simulink model "gm_MATE_HDLsolver_myFirstCircuit"  (R2024b)
settings: Solver=FixedStepDiscrete  StartTime=0.0  StopTime=0.05  FixedStep=6.02409638554217e-09  MaxStep=100e-6  RelTol=1e-4
PostLoadFcn:
  | Ts=1e-6; nb_sw=3; nb_lc=2;nb_r=1;nb_src=1; nb_out=3; rL=1.2;rC=100;L=1e-3; C=1e-5; LpejoSw=1e-6;h=Ts; MAX_INPUTS=16;
  | MAX_OUTPUTS=16;
  | MAX_SWITCHES=8;
  | MAX_INPUTS=16;
InitFcn:
  | Ts=1e-6; nb_sw=3; nb_lc=2;nb_r=1;nb_src=1; nb_out=3; rL=1.2;rC=100;L=1e-3; C=1e-5; LpejoSw=1e-6;h=Ts; MAX_INPUTS=16;
  | MAX_OUTPUTS=16;
  | MAX_SWITCHES=8;
  | MAX_INPUTS=16;
undefined symbols (not defined in the file or in its folder): MATE_SOC
libraries: fl_lib x31, nesl_utility x13, hdlmdlgenlib x10, simetranss x5, simulink x4, hdlsllib x3, ee_lib x2, eeGeneralControl x1
(part 2 of 8)

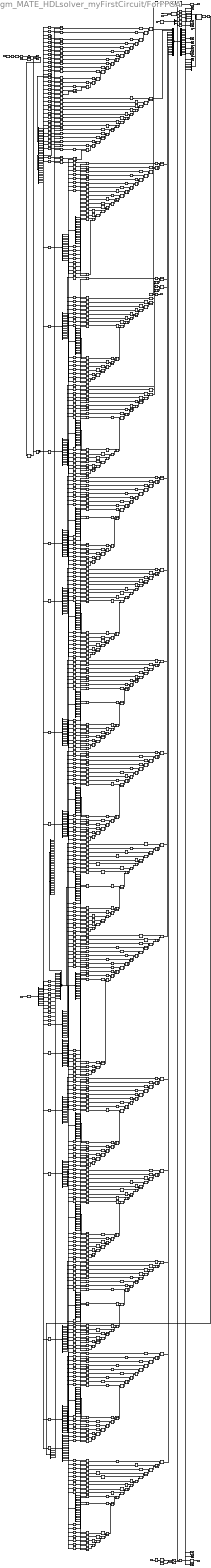
== system gm_MATE_HDLsolver_myFirstCircuit/ForFPGA ==
  note: Pejos
  mi : Inport  OutDataTypeStr=single  PortDimensions=1  SampleTime=1e-06
  PWMsteps : Inport  Port=2  OutDataTypeStr=uint16  PortDimensions=1  SampleTime=1e-06
  gate : Inport  Port=3  OutDataTypeStr=boolean  PortDimensions=[3]  SampleTime=1e-06
  minus_g : Inport  Port=4  OutDataTypeStr=single  PortDimensions=[5]  SampleTime=1e-06
  CrossIC : Inport  Port=5  OutDataTypeStr=boolean  PortDimensions=[5]  SampleTime=1e-06
  CrossICidx : Inport  Port=6  OutDataTypeStr=uint16  PortDimensions=[5]  SampleTime=1e-06
  D : Inport  Port=7  OutDataTypeStr=single  PortDimensions=1  SampleTime=1e-06
  Dcnt : Inport  Port=8  OutDataTypeStr=uint8  PortDimensions=1  SampleTime=1e-06
  in : Inport  Port=9  OutDataTypeStr=single  PortDimensions=[11]  SampleTime=1e-06
  out_start_range : Inport  Port=10  OutDataTypeStr=uint8  PortDimensions=1  SampleTime=1e-06
  Compare To Constant : Subsystem  mask(Compare To Constant){relop===, const=double(0), OutDataTypeStr=boolean, ZeroCross=on}
      mask prompts: relop "Simulink:masks:Operator_MP"; const "Simulink:masks:ConstantValue_MP"; OutDataTypeStr "Simulink:masks:OutputDataType_MP"; ZeroCross "Simulink:masks:EnableZerocrossingDetection_MP"
      mask help: Simulink:masks:CompareToConstant_MD
      mask init:
      | OutDataTypeStr = 'boolean';
      | ZeroCross = 'on';
      | blkName = 'MATE_HDLsolver_myFirstCircuit/ForFPGA/Compare\nTo Constant';
      | const = double(0);
      | const_str = '0';
      | const_val = double(0);
      | relop = '==';
      | setValue = 'boolean';
      | str = '== 0';
      mask TypeOptions relop: == | ~= | < | <= | >= | >
      mask TypeOptions OutDataTypeStr: Simulink:masks:uint8 | Simulink:masks:boolean
      mask Callback ZeroCross: sl('zeroCrossEnable', gcbh);
      mask Display: disp(str)
  Counter Free-Running : Subsystem  mask(Counter Free-Running){NumBits=double(4), tsamp=double(-1)}
      mask prompts: NumBits "Simulink:masks:NumberOfBits_MP"; tsamp "Simulink:masks:SampleTime_MP"
      mask help: Simulink:masks:CounterFreeRunning_MD
  Data Type Conversion1 : DataTypeConversion  OutDataTypeStr=boolean
  Data Type Conversion2 : DataTypeConversion  OutDataTypeStr=boolean
  Delay : RateTransition  InitialCondition=double(0)  OutPortSampleTimeOpt=Multiple of input port sample time  OutPortSampleTimeMultiple=166
  Delay_Switch : Switch  Criteria=u2 ~= 0  Threshold=double(0)  OutDataTypeStr=single  SampleTime=1e-06  SaturateOnIntegerOverflow=off  InputSameDT=off
  Delay_absorbed : Delay  DelayLength=0
  Demux_mux_1 : Mux  Inputs=5
  Dot Product : Subsystem
      mask Display: disp('NFP\nadd');
  Dot Product1 : Subsystem
      mask Display: disp('NFP\nadd');
  Dot Product10 : Subsystem
      mask Display: disp('NFP\nadd');
  Dot Product101 : Subsystem
      mask Display: disp('NFP\nadd');
  Dot Product1010 : Subsystem
      mask Display: disp('NFP\nadd');
  Dot Product1011 : Subsystem
      mask Display: disp('NFP\nadd');
  Dot Product1012 : Subsystem
      mask Display: disp('NFP\nadd');
  Dot Product1013 : Subsystem
      mask Display: disp('NFP\nadd');
  Dot Product1014 : Subsystem
      mask Display: disp('NFP\nadd');
  Dot Product1015 : Subsystem
      mask Display: disp('NFP\nadd');
  Dot Product102 : Subsystem
      mask Display: disp('NFP\nadd');
  Dot Product103 : Subsystem
      mask Display: disp('NFP\nadd');
  Dot Product104 : Subsystem
      mask Display: disp('NFP\nadd');
  Dot Product105 : Subsystem
      mask Display: disp('NFP\nadd');
  Dot Product106 : Subsystem
      mask Display: disp('NFP\nadd');
  Dot Product107 : Subsystem
      mask Display: disp('NFP\nadd');
  Dot Product108 : Subsystem
      mask Display: disp('NFP\nadd');
  Dot Product109 : Subsystem
      mask Display: disp('NFP\nadd');
  Dot Product11 : Subsystem
      mask Display: disp('NFP\nadd');
  Dot Product110 : Subsystem
      mask Display: disp('NFP\nadd');
  Dot Product111 : Subsystem
      mask Display: disp('NFP\nadd');
  Dot Product1110 : Subsystem
      mask Display: disp('NFP\nadd');
  Dot Product1111 : Subsystem
      mask Display: disp('NFP\nadd');
  Dot Product1112 : Subsystem
      mask Display: disp('NFP\nadd');
  Dot Product1113 : Subsystem
      mask Display: disp('NFP\nadd');
  Dot Product1114 : Subsystem
      mask Display: disp('NFP\nadd');
  Dot Product1115 : Subsystem
      mask Display: disp('NFP\nadd');
  Dot Product1116 : Subsystem
      mask Display: disp('NFP\nadd');
  Dot Product1117 : Subsystem
      mask Display: disp('NFP\nadd');
  Dot Product1118 : Subsystem
      mask Display: disp('NFP\nadd');
  Dot Product1119 : Subsystem
      mask Display: disp('NFP\nadd');
  Dot Product112 : Subsystem
      mask Display: disp('NFP\nadd');
  Dot Product1120 : Subsystem
      mask Display: disp('NFP\nadd');
  Dot Product1121 : Subsystem
      mask Display: disp('NFP\nadd');
  Dot Product1122 : Subsystem
      mask Display: disp('NFP\nadd');
  Dot Product1123 : Subsystem
      mask Display: disp('NFP\nadd');
  Dot Product1124 : Subsystem
      mask Display: disp('NFP\nadd');
  Dot Product113 : Subsystem
      mask Display: disp('NFP\nadd');
  Dot Product114 : Subsystem
      mask Display: disp('NFP\nadd');
  Dot Product115 : Subsystem
      mask Display: disp('NFP\nadd');
  Dot Product116 : Subsystem
      mask Display: disp('NFP\nadd');
  Dot Product117 : Subsystem
      mask Display: disp('NFP\nadd');
  Dot Product118 : Subsystem
      mask Display: disp('NFP\nadd');
  Dot Product119 : Subsystem
      mask Display: disp('NFP\nadd');
  Dot Product12 : Subsystem
      mask Display: disp('NFP\nadd');
  Dot Product121 : Subsystem
      mask Display: disp('NFP\nadd');
  Dot Product1210 : Subsystem
      mask Display: disp('NFP\nadd');
  Dot Product1211 : Subsystem
      mask Display: disp('NFP\nadd');
  Dot Product1212 : Subsystem
      mask Display: disp('NFP\nadd');
  Dot Product1213 : Subsystem
      mask Display: disp('NFP\nadd');
  Dot Product1214 : Subsystem
      mask Display: disp('NFP\nadd');
  Dot Product1215 : Subsystem
      mask Display: disp('NFP\nadd');
  Dot Product122 : Subsystem
      mask Display: disp('NFP\nadd');
  Dot Product123 : Subsystem
      mask Display: disp('NFP\nadd');
  Dot Product124 : Subsystem
      mask Display: disp('NFP\nadd');
  Dot Product125 : Subsystem
      mask Display: disp('NFP\nadd');
  Dot Product126 : Subsystem
      mask Display: disp('NFP\nadd');
  Dot Product127 : Subsystem
      mask Display: disp('NFP\nadd');
  Dot Product128 : Subsystem
      mask Display: disp('NFP\nadd');
  Dot Product129 : Subsystem
      mask Display: disp('NFP\nadd');
  Dot Product13 : Subsystem
      mask Display: disp('NFP\nadd');
  Dot Product131 : Subsystem
      mask Display: disp('NFP\nadd');
  Dot Product1310 : Subsystem
      mask Display: disp('NFP\nadd');
  Dot Product1311 : Subsystem
      mask Display: disp('NFP\nadd');
  Dot Product1312 : Subsystem
      mask Display: disp('NFP\nadd');
  Dot Product1313 : Subsystem
      mask Display: disp('NFP\nadd');
  Dot Product1314 : Subsystem
      mask Display: disp('NFP\nadd');
  Dot Product1315 : Subsystem
      mask Display: disp('NFP\nadd');
  Dot Product132 : Subsystem
      mask Display: disp('NFP\nadd');
  Dot Product133 : Subsystem
      mask Display: disp('NFP\nadd');
  Dot Product134 : Subsystem
      mask Display: disp('NFP\nadd');
  Dot Product135 : Subsystem
      mask Display: disp('NFP\nadd');
  Dot Product136 : Subsystem
      mask Display: disp('NFP\nadd');
  Dot Product137 : Subsystem
      mask Display: disp('NFP\nadd');
  Dot Product138 : Subsystem
      mask Display: disp('NFP\nadd');
  Dot Product139 : Subsystem
      mask Display: disp('NFP\nadd');
  Dot Product14 : Subsystem
      mask Display: disp('NFP\nadd');
  Dot Product141 : Subsystem
      mask Display: disp('NFP\nadd');
  Dot Product1410 : Subsystem
      mask Display: disp('NFP\nadd');
  Dot Product1411 : Subsystem
      mask Display: disp('NFP\nadd');
  Dot Product1412 : Subsystem
      mask Display: disp('NFP\nadd');
  Dot Product1413 : Subsystem
      mask Display: disp('NFP\nadd');
  Dot Product1414 : Subsystem
      mask Display: disp('NFP\nadd');
  Dot Product1415 : Subsystem
      mask Display: disp('NFP\nadd');
  Dot Product142 : Subsystem
      mask Display: disp('NFP\nadd');
  Dot Product143 : Subsystem
      mask Display: disp('NFP\nadd');
  Dot Product144 : Subsystem
      mask Display: disp('NFP\nadd');
  Dot Product145 : Subsystem
      mask Display: disp('NFP\nadd');
  Dot Product146 : Subsystem
      mask Display: disp('NFP\nadd');
  Dot Product147 : Subsystem
      mask Display: disp('NFP\nadd');
  Dot Product148 : Subsystem
      mask Display: disp('NFP\nadd');
  Dot Product149 : Subsystem
      mask Display: disp('NFP\nadd');
  Dot Product15 : Subsystem
      mask Display: disp('NFP\nadd');
  Dot Product151 : Subsystem
      mask Display: disp('NFP\nadd');
  Dot Product1510 : Subsystem
      mask Display: disp('NFP\nadd');
  Dot Product1511 : Subsystem
      mask Display: disp('NFP\nadd');
  Dot Product1512 : Subsystem
      mask Display: disp('NFP\nadd');
  Dot Product1513 : Subsystem
      mask Display: disp('NFP\nadd');
  Dot Product1514 : Subsystem
      mask Display: disp('NFP\nadd');
  Dot Product1515 : Subsystem
      mask Display: disp('NFP\nadd');
  Dot Product152 : Subsystem
      mask Display: disp('NFP\nadd');
  Dot Product153 : Subsystem
      mask Display: disp('NFP\nadd');
  Dot Product154 : Subsystem
      mask Display: disp('NFP\nadd');
  Dot Product155 : Subsystem
      mask Display: disp('NFP\nadd');
  Dot Product156 : Subsystem
      mask Display: disp('NFP\nadd');
  Dot Product157 : Subsystem
      mask Display: disp('NFP\nadd');
  Dot Product158 : Subsystem
      mask Display: disp('NFP\nadd');
  Dot Product159 : Subsystem
      mask Display: disp('NFP\nadd');
  Dot Product16 : Subsystem
      mask Display: disp('NFP\nadd');
  Dot Product17 : Subsystem
      mask Display: disp('NFP\nadd');
  Dot Product18 : Subsystem
      mask Display: disp('NFP\nadd');
  Dot Product19 : Subsystem
      mask Display: disp('NFP\nadd');
  Dot Product2 : Subsystem
      mask Display: disp('NFP\nadd');
  Dot Product21 : Subsystem
      mask Display: disp('NFP\nadd');
  Dot Product210 : Subsystem
      mask Display: disp('NFP\nadd');
  Dot Product211 : Subsystem
      mask Display: disp('NFP\nadd');
  Dot Product212 : Subsystem
      mask Display: disp('NFP\nadd');
  Dot Product213 : Subsystem
      mask Display: disp('NFP\nadd');
  Dot Product214 : Subsystem
      mask Display: disp('NFP\nadd');
  Dot Product215 : Subsystem
      mask Display: disp('NFP\nadd');
  Dot Product22 : Subsystem
      mask Display: disp('NFP\nadd');
  Dot Product23 : Subsystem
      mask Display: disp('NFP\nadd');
  Dot Product24 : Subsystem
      mask Display: disp('NFP\nadd');
  Dot Product25 : Subsystem
      mask Display: disp('NFP\nadd');
  Dot Product26 : Subsystem
      mask Display: disp('NFP\nadd');
  Dot Product27 : Subsystem
      mask Display: disp('NFP\nadd');
  Dot Product28 : Subsystem
      mask Display: disp('NFP\nadd');
  Dot Product29 : Subsystem
      mask Display: disp('NFP\nadd');
  Dot Product3 : Subsystem
      mask Display: disp('NFP\nadd');
  Dot Product31 : Subsystem
      mask Display: disp('NFP\nadd');
  Dot Product310 : Subsystem
      mask Display: disp('NFP\nadd');
  Dot Product311 : Subsystem
      mask Display: disp('NFP\nadd');
  Dot Product312 : Subsystem
      mask Display: disp('NFP\nadd');
  Dot Product313 : Subsystem
      mask Display: disp('NFP\nadd');
  Dot Product314 : Subsystem
      mask Display: disp('NFP\nadd');
  Dot Product315 : Subsystem
      mask Display: disp('NFP\nadd');
  Dot Product32 : Subsystem
      mask Display: disp('NFP\nadd');
  Dot Product33 : Subsystem
      mask Display: disp('NFP\nadd');
  Dot Product34 : Subsystem
      mask Display: disp('NFP\nadd');
  Dot Product35 : Subsystem
      mask Display: disp('NFP\nadd');
  Dot Product36 : Subsystem
      mask Display: disp('NFP\nadd');
  Dot Product37 : Subsystem
      mask Display: disp('NFP\nadd');
  Dot Product38 : Subsystem
      mask Display: disp('NFP\nadd');
  Dot Product39 : Subsystem
      mask Display: disp('NFP\nadd');
  Dot Product4 : Subsystem
      mask Display: disp('NFP\nadd');
  Dot Product41 : Subsystem
      mask Display: disp('NFP\nadd');
  Dot Product410 : Subsystem
      mask Display: disp('NFP\nadd');
  Dot Product411 : Subsystem
      mask Display: disp('NFP\nadd');
  Dot Product412 : Subsystem
      mask Display: disp('NFP\nadd');
  Dot Product413 : Subsystem
      mask Display: disp('NFP\nadd');
  Dot Product414 : Subsystem
      mask Display: disp('NFP\nadd');
  Dot Product415 : Subsystem
      mask Display: disp('NFP\nadd');
  Dot Product42 : Subsystem
      mask Display: disp('NFP\nadd');
  Dot Product43 : Subsystem
      mask Display: disp('NFP\nadd');
  Dot Product44 : Subsystem
      mask Display: disp('NFP\nadd');
  Dot Product45 : Subsystem
      mask Display: disp('NFP\nadd');
  Dot Product46 : Subsystem
      mask Display: disp('NFP\nadd');
  Dot Product47 : Subsystem
      mask Display: disp('NFP\nadd');
  Dot Product48 : Subsystem
      mask Display: disp('NFP\nadd');
  Dot Product49 : Subsystem
      mask Display: disp('NFP\nadd');
  Dot Product5 : Subsystem
      mask Display: disp('NFP\nadd');
  Dot Product51 : Subsystem
      mask Display: disp('NFP\nadd');
  Dot Product510 : Subsystem
      mask Display: disp('NFP\nadd');
  Dot Product511 : Subsystem
      mask Display: disp('NFP\nadd');
  Dot Product512 : Subsystem
      mask Display: disp('NFP\nadd');
  Dot Product513 : Subsystem
      mask Display: disp('NFP\nadd');
  Dot Product514 : Subsystem
      mask Display: disp('NFP\nadd');
  Dot Product515 : Subsystem
      mask Display: disp('NFP\nadd');
  Dot Product52 : Subsystem
      mask Display: disp('NFP\nadd');
  Dot Product53 : Subsystem
      mask Display: disp('NFP\nadd');
  Dot Product54 : Subsystem
      mask Display: disp('NFP\nadd');
  Dot Product55 : Subsystem
      mask Display: disp('NFP\nadd');
  Dot Product56 : Subsystem
      mask Display: disp('NFP\nadd');
  Dot Product57 : Subsystem
      mask Display: disp('NFP\nadd');
  Dot Product58 : Subsystem
      mask Display: disp('NFP\nadd');
  Dot Product59 : Subsystem
      mask Display: disp('NFP\nadd');
  Dot Product6 : Subsystem
      mask Display: disp('NFP\nadd');
  Dot Product61 : Subsystem
      mask Display: disp('NFP\nadd');
  Dot Product610 : Subsystem
      mask Display: disp('NFP\nadd');
  Dot Product611 : Subsystem
      mask Display: disp('NFP\nadd');
  Dot Product612 : Subsystem
      mask Display: disp('NFP\nadd');
  Dot Product613 : Subsystem
      mask Display: disp('NFP\nadd');
  Dot Product614 : Subsystem
      mask Display: disp('NFP\nadd');
  Dot Product615 : Subsystem
      mask Display: disp('NFP\nadd');
  Dot Product62 : Subsystem
      mask Display: disp('NFP\nadd');
  Dot Product63 : Subsystem
      mask Display: disp('NFP\nadd');
  Dot Product64 : Subsystem
      mask Display: disp('NFP\nadd');
  Dot Product65 : Subsystem
      mask Display: disp('NFP\nadd');
  Dot Product66 : Subsystem
      mask Display: disp('NFP\nadd');
  Dot Product67 : Subsystem
      mask Display: disp('NFP\nadd');
  Dot Product68 : Subsystem
      mask Display: disp('NFP\nadd');
  Dot Product69 : Subsystem
      mask Display: disp('NFP\nadd');
  Dot Product7 : Subsystem
      mask Display: disp('NFP\nadd');
  Dot Product71 : Subsystem
      mask Display: disp('NFP\nadd');
  Dot Product710 : Subsystem
      mask Display: disp('NFP\nadd');
  Dot Product711 : Subsystem
      mask Display: disp('NFP\nadd');
  Dot Product712 : Subsystem
      mask Display: disp('NFP\nadd');
  Dot Product713 : Subsystem
      mask Display: disp('NFP\nadd');
  Dot Product714 : Subsystem
      mask Display: disp('NFP\nadd');
  Dot Product715 : Subsystem
      mask Display: disp('NFP\nadd');
  Dot Product72 : Subsystem
      mask Display: disp('NFP\nadd');
  Dot Product73 : Subsystem
      mask Display: disp('NFP\nadd');
  Dot Product74 : Subsystem
      mask Display: disp('NFP\nadd');
  Dot Product75 : Subsystem
      mask Display: disp('NFP\nadd');
  Dot Product76 : Subsystem
      mask Display: disp('NFP\nadd');
  Dot Product77 : Subsystem
      mask Display: disp('NFP\nadd');
  Dot Product78 : Subsystem
      mask Display: disp('NFP\nadd');
  Dot Product79 : Subsystem
      mask Display: disp('NFP\nadd');
  Dot Product8 : Subsystem
      mask Display: disp('NFP\nadd');
  Dot Product81 : Subsystem
      mask Display: disp('NFP\nadd');
  Dot Product810 : Subsystem
      mask Display: disp('NFP\nadd');
  Dot Product811 : Subsystem
      mask Display: disp('NFP\nadd');
  Dot Product812 : Subsystem
      mask Display: disp('NFP\nadd');
  Dot Product813 : Subsystem
      mask Display: disp('NFP\nadd');
  Dot Product814 : Subsystem
      mask Display: disp('NFP\nadd');
  Dot Product815 : Subsystem
      mask Display: disp('NFP\nadd');
  Dot Product82 : Subsystem
      mask Display: disp('NFP\nadd');
  Dot Product83 : Subsystem
      mask Display: disp('NFP\nadd');
  Dot Product84 : Subsystem
      mask Display: disp('NFP\nadd');
  Dot Product85 : Subsystem
      mask Display: disp('NFP\nadd');
  Dot Product86 : Subsystem
      mask Display: disp('NFP\nadd');
  Dot Product87 : Subsystem
      mask Display: disp('NFP\nadd');
  Dot Product88 : Subsystem
      mask Display: disp('NFP\nadd');
  Dot Product89 : Subsystem
      mask Display: disp('NFP\nadd');
  Dot Product9 : Subsystem
      mask Display: disp('NFP\nadd');
  Dot Product91 : Subsystem
      mask Display: disp('NFP\nadd');
  Dot Product910 : Subsystem
      mask Display: disp('NFP\nadd');
  Dot Product911 : Subsystem
      mask Display: disp('NFP\nadd');
  Dot Product912 : Subsystem
      mask Display: disp('NFP\nadd');
  Dot Product913 : Subsystem
      mask Display: disp('NFP\nadd');
  Dot Product914 : Subsystem
      mask Display: disp('NFP\nadd');
  Dot Product915 : Subsystem
      mask Display: disp('NFP\nadd');
  Dot Product92 : Subsystem
      mask Display: disp('NFP\nadd');
  Dot Product93 : Subsystem
      mask Display: disp('NFP\nadd');
  Dot Product94 : Subsystem
      mask Display: disp('NFP\nadd');
  Dot Product95 : Subsystem
      mask Display: disp('NFP\nadd');
  Dot Product96 : Subsystem
      mask Display: disp('NFP\nadd');
  Dot Product97 : Subsystem
      mask Display: disp('NFP\nadd');
  Dot Product98 : Subsystem
      mask Display: disp('NFP\nadd');
  Dot Product99 : Subsystem
      mask Display: disp('NFP\nadd');
  From : hdlmdlgenlib/Buffer
  Goto : hdlmdlgenlib/Buffer
  Index Vector : MultiPortSwitch  DataPortOrder=Zero-based contiguous  Inputs=1  DiagnosticForDefault=None  zeroidx=on  OutDataTypeStr=single  SampleTime=6.02409638554217e-09  SaturateOnIntegerOverflow=off  InputSameDT=off
  Index Vector_dtc_comp : DataTypeConversion  OutDataTypeStr=fixdt(0, 4, 0)  SampleTime=6.02409638554217e-09  SaturateOnIntegerOverflow=off
  LC vectorized : Subsystem
  Mux4_out1_10_term10 : Terminator
  Mux4_out1_11_term11 : Terminator
  Mux4_out1_12_term12 : Terminator
  Mux4_out1_13_term13 : Terminator
  Mux4_out1_14_term14 : Terminator
  Mux4_out1_15_term15 : Terminator
  Mux4_out1_5_term5 : Terminator
  Mux4_out1_6_term6 : Terminator
  Mux4_out1_7_term7 : Terminator
  Mux4_out1_8_term8 : Terminator
  Mux4_out1_9_term9 : Terminator
  PWM Generator : Subsystem
  Selector : Selector  InputPortWidth=256  IndexOptions=Index vector (dialog)  Indices=double([1 2 3 4 5 6 7 8 9 10 11 12 13 14 15 16])  OutputSizes=double(1)
  Selector1 : Selector  InputPortWidth=256  IndexOptions=Index vector (dialog)  Indices=double([17 18 19 20 21 22 23 24 25 26 27 28 29 30 31 32])  OutputSizes=double(1)
  Selector10 : Selector  InputPortWidth=256  IndexOptions=Index vector (dialog)  Indices=double([161 162 163 164 165 166 167 168 169 170 171 172 173 174 175 176])  OutputSizes=double(1)
  Selector11 : Selector  InputPortWidth=256  IndexOptions=Index vector (dialog)  Indices=double([177 178 179 180 181 182 183 184 185 186 187 188 189 190 191 192])  OutputSizes=double(1)
  Selector12 : Selector  InputPortWidth=256  IndexOptions=Index vector (dialog)  Indices=double([193 194 195 196 197 198 199 200 201 202 203 204 205 206 207 208])  OutputSizes=double(1)
  Selector13 : Selector  InputPortWidth=256  IndexOptions=Index vector (dialog)  Indices=double([209 210 211 212 213 214 215 216 217 218 219 220 221 222 223 224])  OutputSizes=double(1)
  Selector14 : Selector  InputPortWidth=256  IndexOptions=Index vector (dialog)  Indices=double([225 226 227 228 229 230 231 232 233 234 235 236 237 238 239 240])  OutputSizes=double(1)
  Selector15 : Selector  InputPortWidth=256  IndexOptions=Index vector (dialog)  Indices=double([241 242 243 244 245 246 247 248 249 250 251 252 253 254 255 256])  OutputSizes=double(1)
  Selector16 : Selector  InputPortWidth=16  IndexOptions=Starting index (port)  Indices=double([1 2 3 4 5 6 7 8 9 10 11 12 13 14 15 16])  OutputSizes=double(8)
  Selector2 : Selector  InputPortWidth=256  IndexOptions=Index vector (dialog)  Indices=double([33 34 35 36 37 38 39 40 41 42 43 44 45 46 47 48])  OutputSizes=double(1)
  Selector3 : Selector  InputPortWidth=256  IndexOptions=Index vector (dialog)  Indices=double([49 50 51 52 53 54 55 56 57 58 59 60 61 62 63 64])  OutputSizes=double(1)
  Selector4 : Selector  InputPortWidth=256  IndexOptions=Index vector (dialog)  Indices=double([65 66 67 68 69 70 71 72 73 74 75 76 77 78 79 80])  OutputSizes=double(1)
  Selector5 : Selector  InputPortWidth=256  IndexOptions=Index vector (dialog)  Indices=double([81 82 83 84 85 86 87 88 89 90 91 92 93 94 95 96])  OutputSizes=double(1)
  Selector6 : Selector  InputPortWidth=256  IndexOptions=Index vector (dialog)  Indices=double([97 98 99 100 101 102 103 104 105 106 107 108 109 110 111 112])  OutputSizes=double(1)
  Selector7 : Selector  InputPortWidth=256  IndexOptions=Index vector (dialog)  Indices=double([113 114 115 116 117 118 119 120 121 122 123 124 125 126 127 128])  OutputSizes=double(1)
  Selector8 : Selector  InputPortWidth=256  IndexOptions=Index vector (dialog)  Indices=double([129 130 131 132 133 134 135 136 137 138 139 140 141 142 143 144])  OutputSizes=double(1)
  Selector9 : Selector  InputPortWidth=256  IndexOptions=Index vector (dialog)  Indices=double([145 146 147 148 149 150 151 152 153 154 155 156 157 158 159 160])  OutputSizes=double(1)
  Tapped Delay : simulink/Discrete/Tapped Delay  vinit=0  samptime=-1  NumDelays=double(255)  DelayOrder=Oldest  includeCurrent=on
  Unit Delay Enabled Synchronous22_lowered : Delay  DelayLength=double(1)  InitialCondition=0  SampleTime=1e-06
  crp_out_delay : Delay  DelayLength=double(1)  InitialCondition=0  SampleTime=6.02409638554217e-09
  delayMatch{,1..29,33,44..59,63,74..89,93,104..119,123,134..149,153,164..179,183,194..209,213,224..239,243,254..269,273,284..299,303,314..329,333,344..359,363,374..389,393,404..419,423,434..449,453,464..479,483} (286 alike) : Delay  DelayLength=double(24)  InitialCondition=0  SampleTime=6.02409638554217e-09
  delayMatch{40,70,100,130,160,190,220,250,280,310,340,370,400,430,460,490} (16 alike) : Delay  DelayLength=double(66)  InitialCondition=0  SampleTime=6.02409638554217e-09
  delayMatch{41,71,101,131,161,191,221,251,281,311,341,371,401,431,461,491} (16 alike) : Delay  DelayLength=double(72)  InitialCondition=0  SampleTime=6.02409638554217e-09
  delayMatch{42,72,102,132,162,192,222,252,282,312,342,372,402,432,462,492} (16 alike) : Delay  DelayLength=double(78)  InitialCondition=0  SampleTime=6.02409638554217e-09
  delayMatch{43,73,103,133,163,193,223,253,283,313,343,373,403,433,463,493} (16 alike) : Delay  DelayLength=double(84)  InitialCondition=0  SampleTime=6.02409638554217e-09
  delayMatch{30,60,90,120,150,180,210,240,270,300,330,360,390,420,450,480} (16 alike) : Delay  DelayLength=double(6)  InitialCondition=0  SampleTime=6.02409638554217e-09
  delayMatch{31,61,91,121,151,181,211,241,271,301,331,361,391,421,451,481} (16 alike) : Delay  DelayLength=double(12)  InitialCondition=0  SampleTime=6.02409638554217e-09
  delayMatch{32,62,92,122,152,182,212,242,272,302,332,362,392,422,452,482} (16 alike) : Delay  DelayLength=double(18)  InitialCondition=0  SampleTime=6.02409638554217e-09
  delayMatch{34,64,94,124,154,184,214,244,274,304,334,364,394,424,454,484} (16 alike) : Delay  DelayLength=double(30)  InitialCondition=0  SampleTime=6.02409638554217e-09
  delayMatch{35,65,95,125,155,185,215,245,275,305,335,365,395,425,455,485} (16 alike) : Delay  DelayLength=double(36)  InitialCondition=0  SampleTime=6.02409638554217e-09
  delayMatch{36,66,96,126,156,186,216,246,276,306,336,366,396,426,456,486} (16 alike) : Delay  DelayLength=double(42)  InitialCondition=0  SampleTime=6.02409638554217e-09
  delayMatch{37,67,97,127,157,187,217,247,277,307,337,367,397,427,457,487} (16 alike) : Delay  DelayLength=double(48)  InitialCondition=0  SampleTime=6.02409638554217e-09
  delayMatch{38,68,98,128,158,188,218,248,278,308,338,368,398,428,458,488} (16 alike) : Delay  DelayLength=double(54)  InitialCondition=0  SampleTime=6.02409638554217e-09
  delayMatch{39,69,99,129,159,189,219,249,279,309,339,369,399,429,459,489} (16 alike) : Delay  DelayLength=double(60)  InitialCondition=0  SampleTime=6.02409638554217e-09
  delayMatch494 : Delay  DelayLength=double(1)  InitialCondition=0  SampleTime=6.02409638554217e-09
  delayMatch495 : Delay  DelayLength=double(1)  InitialCondition=0  SampleTime=6.02409638554217e-09
  delayMatch496 : Delay  DelayLength=double(1)  InitialCondition=0  SampleTime=1e-06
  in0_repeat : RateTransition  Integrity=off  Deterministic=off  OutPortSampleTimeOpt=Multiple of input port sample time  OutPortSampleTimeMultiple=1/166
  in1_repeat : RateTransition  Integrity=off  Deterministic=off  OutPortSampleTimeOpt=Multiple of input port sample time  OutPortSampleTimeMultiple=1/166
  in2_repeat : RateTransition  Integrity=off  Deterministic=off  OutPortSampleTimeOpt=Multiple of input port sample time  OutPortSampleTimeMultiple=1/166
  in3_repeat : RateTransition  Integrity=off  Deterministic=off  OutPortSampleTimeOpt=Multiple of input port sample time  OutPortSampleTimeMultiple=1/166
  in3_repeat1 : RateTransition  Integrity=off  Deterministic=off  OutPortSampleTimeOpt=Multiple of input port sample time  OutPortSampleTimeMultiple=1/166
  in4_repeat : RateTransition  Integrity=off  Deterministic=off  OutPortSampleTimeOpt=Multiple of input port sample time  OutPortSampleTimeMultiple=1/166
  mul_Dot Product10_dotp_0 : Subsystem
      mask Display: disp('NFP\nmul');
  mul_Dot Product10_dotp_1 : Subsystem
      mask Display: disp('NFP\nmul');
  mul_Dot Product10_dotp_10 : Subsystem
      mask Display: disp('NFP\nmul');
  mul_Dot Product10_dotp_11 : Subsystem
      mask Display: disp('NFP\nmul');
  mul_Dot Product10_dotp_12 : Subsystem
      mask Display: disp('NFP\nmul');
  mul_Dot Product10_dotp_13 : Subsystem
      mask Display: disp('NFP\nmul');
  mul_Dot Product10_dotp_14 : Subsystem
      mask Display: disp('NFP\nmul');
  mul_Dot Product10_dotp_15 : Subsystem
      mask Display: disp('NFP\nmul');
  mul_Dot Product10_dotp_2 : Subsystem
      mask Display: disp('NFP\nmul');
  mul_Dot Product10_dotp_3 : Subsystem
      mask Display: disp('NFP\nmul');
  mul_Dot Product10_dotp_4 : Subsystem
      mask Display: disp('NFP\nmul');
  mul_Dot Product10_dotp_5 : Subsystem
      mask Display: disp('NFP\nmul');
  mul_Dot Product10_dotp_6 : Subsystem
      mask Display: disp('NFP\nmul');
  mul_Dot Product10_dotp_7 : Subsystem
      mask Display: disp('NFP\nmul');
  mul_Dot Product10_dotp_8 : Subsystem
      mask Display: disp('NFP\nmul');
  mul_Dot Product10_dotp_9 : Subsystem
      mask Display: disp('NFP\nmul');
  mul_Dot Product11_dotp_0 : Subsystem
      mask Display: disp('NFP\nmul');
  mul_Dot Product11_dotp_1 : Subsystem
      mask Display: disp('NFP\nmul');
  mul_Dot Product11_dotp_10 : Subsystem
      mask Display: disp('NFP\nmul');
  mul_Dot Product11_dotp_11 : Subsystem
      mask Display: disp('NFP\nmul');
  mul_Dot Product11_dotp_12 : Subsystem
      mask Display: disp('NFP\nmul');
  mul_Dot Product11_dotp_13 : Subsystem
      mask Display: disp('NFP\nmul');
  mul_Dot Product11_dotp_14 : Subsystem
      mask Display: disp('NFP\nmul');
  mul_Dot Product11_dotp_15 : Subsystem
      mask Display: disp('NFP\nmul');
  mul_Dot Product11_dotp_2 : Subsystem
      mask Display: disp('NFP\nmul');
  mul_Dot Product11_dotp_3 : Subsystem
      mask Display: disp('NFP\nmul');
  mul_Dot Product11_dotp_4 : Subsystem
      mask Display: disp('NFP\nmul');
  mul_Dot Product11_dotp_5 : Subsystem
      mask Display: disp('NFP\nmul');
  mul_Dot Product11_dotp_6 : Subsystem
      mask Display: disp('NFP\nmul');
  mul_Dot Product11_dotp_7 : Subsystem
      mask Display: disp('NFP\nmul');
  mul_Dot Product11_dotp_8 : Subsystem
      mask Display: disp('NFP\nmul');
  mul_Dot Product11_dotp_9 : Subsystem
      mask Display: disp('NFP\nmul');
  mul_Dot Product12_dotp_0 : Subsystem
      mask Display: disp('NFP\nmul');
  mul_Dot Product12_dotp_1 : Subsystem
      mask Display: disp('NFP\nmul');
  mul_Dot Product12_dotp_10 : Subsystem
      mask Display: disp('NFP\nmul');
  mul_Dot Product12_dotp_11 : Subsystem
      mask Display: disp('NFP\nmul');
  mul_Dot Product12_dotp_12 : Subsystem
      mask Display: disp('NFP\nmul');
  mul_Dot Product12_dotp_13 : Subsystem
      mask Display: disp('NFP\nmul');
  mul_Dot Product12_dotp_14 : Subsystem
      mask Display: disp('NFP\nmul');
  mul_Dot Product12_dotp_15 : Subsystem
      mask Display: disp('NFP\nmul');
  mul_Dot Product12_dotp_2 : Subsystem
      mask Display: disp('NFP\nmul');
  mul_Dot Product12_dotp_3 : Subsystem
      mask Display: disp('NFP\nmul');
  mul_Dot Product12_dotp_4 : Subsystem
      mask Display: disp('NFP\nmul');
  mul_Dot Product12_dotp_5 : Subsystem
      mask Display: disp('NFP\nmul');
  mul_Dot Product12_dotp_6 : Subsystem
      mask Display: disp('NFP\nmul');
  mul_Dot Product12_dotp_7 : Subsystem
      mask Display: disp('NFP\nmul');
  mul_Dot Product12_dotp_8 : Subsystem
      mask Display: disp('NFP\nmul');
  mul_Dot Product12_dotp_9 : Subsystem
      mask Display: disp('NFP\nmul');
  mul_Dot Product13_dotp_0 : Subsystem
      mask Display: disp('NFP\nmul');
  mul_Dot Product13_dotp_1 : Subsystem
      mask Display: disp('NFP\nmul');
  mul_Dot Product13_dotp_10 : Subsystem
      mask Display: disp('NFP\nmul');
  mul_Dot Product13_dotp_11 : Subsystem
      mask Display: disp('NFP\nmul');
  mul_Dot Product13_dotp_12 : Subsystem
      mask Display: disp('NFP\nmul');
  mul_Dot Product13_dotp_13 : Subsystem
      mask Display: disp('NFP\nmul');
  mul_Dot Product13_dotp_14 : Subsystem
      mask Display: disp('NFP\nmul');
  mul_Dot Product13_dotp_15 : Subsystem
      mask Display: disp('NFP\nmul');
  mul_Dot Product13_dotp_2 : Subsystem
      mask Display: disp('NFP\nmul');
  mul_Dot Product13_dotp_3 : Subsystem
      mask Display: disp('NFP\nmul');
  mul_Dot Product13_dotp_4 : Subsystem
      mask Display: disp('NFP\nmul');
  mul_Dot Product13_dotp_5 : Subsystem
      mask Display: disp('NFP\nmul');
  mul_Dot Product13_dotp_6 : Subsystem
      mask Display: disp('NFP\nmul');
  mul_Dot Product13_dotp_7 : Subsystem
      mask Display: disp('NFP\nmul');
  mul_Dot Product13_dotp_8 : Subsystem
      mask Display: disp('NFP\nmul');
  mul_Dot Product13_dotp_9 : Subsystem
      mask Display: disp('NFP\nmul');
  mul_Dot Product14_dotp_0 : Subsystem
      mask Display: disp('NFP\nmul');
  mul_Dot Product14_dotp_1 : Subsystem
      mask Display: disp('NFP\nmul');
  mul_Dot Product14_dotp_10 : Subsystem
      mask Display: disp('NFP\nmul');
  mul_Dot Product14_dotp_11 : Subsystem
      mask Display: disp('NFP\nmul');
  mul_Dot Product14_dotp_12 : Subsystem
      mask Display: disp('NFP\nmul');
  mul_Dot Product14_dotp_13 : Subsystem
      mask Display: disp('NFP\nmul');
  mul_Dot Product14_dotp_14 : Subsystem
      mask Display: disp('NFP\nmul');
  mul_Dot Product14_dotp_15 : Subsystem
      mask Display: disp('NFP\nmul');
  mul_Dot Product14_dotp_2 : Subsystem
      mask Display: disp('NFP\nmul');
  mul_Dot Product14_dotp_3 : Subsystem
      mask Display: disp('NFP\nmul');
  mul_Dot Product14_dotp_4 : Subsystem
      mask Display: disp('NFP\nmul');
  mul_Dot Product14_dotp_5 : Subsystem
      mask Display: disp('NFP\nmul');
  mul_Dot Product14_dotp_6 : Subsystem
      mask Display: disp('NFP\nmul');
  mul_Dot Product14_dotp_7 : Subsystem
      mask Display: disp('NFP\nmul');
  mul_Dot Product14_dotp_8 : Subsystem
      mask Display: disp('NFP\nmul');
  mul_Dot Product14_dotp_9 : Subsystem
      mask Display: disp('NFP\nmul');
  mul_Dot Product15_dotp_0 : Subsystem
      mask Display: disp('NFP\nmul');
  mul_Dot Product15_dotp_1 : Subsystem
      mask Display: disp('NFP\nmul');
  mul_Dot Product15_dotp_10 : Subsystem
      mask Display: disp('NFP\nmul');
  mul_Dot Product15_dotp_11 : Subsystem
      mask Display: disp('NFP\nmul');
  mul_Dot Product15_dotp_12 : Subsystem
      mask Display: disp('NFP\nmul');
  mul_Dot Product15_dotp_13 : Subsystem
      mask Display: disp('NFP\nmul');
  mul_Dot Product15_dotp_14 : Subsystem
      mask Display: disp('NFP\nmul');
  mul_Dot Product15_dotp_15 : Subsystem
      mask Display: disp('NFP\nmul');
  mul_Dot Product15_dotp_2 : Subsystem
      mask Display: disp('NFP\nmul');
  mul_Dot Product15_dotp_3 : Subsystem
      mask Display: disp('NFP\nmul');
  mul_Dot Product15_dotp_4 : Subsystem
      mask Display: disp('NFP\nmul');
  mul_Dot Product15_dotp_5 : Subsystem
      mask Display: disp('NFP\nmul');
  mul_Dot Product15_dotp_6 : Subsystem
      mask Display: disp('NFP\nmul');
  mul_Dot Product15_dotp_7 : Subsystem
      mask Display: disp('NFP\nmul');
  mul_Dot Product15_dotp_8 : Subsystem
      mask Display: disp('NFP\nmul');
  mul_Dot Product15_dotp_9 : Subsystem
      mask Display: disp('NFP\nmul');
  mul_Dot Product1_dotp_0 : Subsystem
      mask Display: disp('NFP\nmul');
  mul_Dot Product1_dotp_1 : Subsystem
      mask Display: disp('NFP\nmul');
  mul_Dot Product1_dotp_10 : Subsystem
      mask Display: disp('NFP\nmul');
  mul_Dot Product1_dotp_11 : Subsystem
      mask Display: disp('NFP\nmul');
  mul_Dot Product1_dotp_12 : Subsystem
      mask Display: disp('NFP\nmul');
  mul_Dot Product1_dotp_13 : Subsystem
      mask Display: disp('NFP\nmul');
  mul_Dot Product1_dotp_14 : Subsystem
      mask Display: disp('NFP\nmul');
  mul_Dot Product1_dotp_15 : Subsystem
      mask Display: disp('NFP\nmul');
  mul_Dot Product1_dotp_2 : Subsystem
      mask Display: disp('NFP\nmul');
  mul_Dot Product1_dotp_3 : Subsystem
      mask Display: disp('NFP\nmul');
  mul_Dot Product1_dotp_4 : Subsystem
      mask Display: disp('NFP\nmul');
  mul_Dot Product1_dotp_5 : Subsystem
      mask Display: disp('NFP\nmul');
  mul_Dot Product1_dotp_6 : Subsystem
      mask Display: disp('NFP\nmul');
  mul_Dot Product1_dotp_7 : Subsystem
      mask Display: disp('NFP\nmul');
  mul_Dot Product1_dotp_8 : Subsystem
      mask Display: disp('NFP\nmul');
  mul_Dot Product1_dotp_9 : Subsystem
      mask Display: disp('NFP\nmul');
  mul_Dot Product2_dotp_0 : Subsystem
      mask Display: disp('NFP\nmul');
  mul_Dot Product2_dotp_1 : Subsystem
      mask Display: disp('NFP\nmul');
  mul_Dot Product2_dotp_10 : Subsystem
      mask Display: disp('NFP\nmul');
  mul_Dot Product2_dotp_11 : Subsystem
      mask Display: disp('NFP\nmul');
  mul_Dot Product2_dotp_12 : Subsystem
      mask Display: disp('NFP\nmul');
  mul_Dot Product2_dotp_13 : Subsystem
      mask Display: disp('NFP\nmul');
  mul_Dot Product2_dotp_14 : Subsystem
      mask Display: disp('NFP\nmul');
  mul_Dot Product2_dotp_15 : Subsystem
      mask Display: disp('NFP\nmul');
  mul_Dot Product2_dotp_2 : Subsystem
      mask Display: disp('NFP\nmul');
  mul_Dot Product2_dotp_3 : Subsystem
      mask Display: disp('NFP\nmul');
  mul_Dot Product2_dotp_4 : Subsystem
      mask Display: disp('NFP\nmul');
  mul_Dot Product2_dotp_5 : Subsystem
      mask Display: disp('NFP\nmul');
  mul_Dot Product2_dotp_6 : Subsystem
      mask Display: disp('NFP\nmul');
  mul_Dot Product2_dotp_7 : Subsystem
      mask Display: disp('NFP\nmul');
  mul_Dot Product2_dotp_8 : Subsystem
      mask Display: disp('NFP\nmul');
  mul_Dot Product2_dotp_9 : Subsystem
      mask Display: disp('NFP\nmul');
  mul_Dot Product3_dotp_0 : Subsystem
      mask Display: disp('NFP\nmul');
  mul_Dot Product3_dotp_1 : Subsystem
      mask Display: disp('NFP\nmul');
  mul_Dot Product3_dotp_10 : Subsystem
      mask Display: disp('NFP\nmul');
  mul_Dot Product3_dotp_11 : Subsystem
      mask Display: disp('NFP\nmul');
  mul_Dot Product3_dotp_12 : Subsystem
      mask Display: disp('NFP\nmul');
  mul_Dot Product3_dotp_13 : Subsystem
      mask Display: disp('NFP\nmul');
  mul_Dot Product3_dotp_14 : Subsystem
      mask Display: disp('NFP\nmul');
  mul_Dot Product3_dotp_15 : Subsystem
      mask Display: disp('NFP\nmul');
  mul_Dot Product3_dotp_2 : Subsystem
      mask Display: disp('NFP\nmul');
  mul_Dot Product3_dotp_3 : Subsystem
      mask Display: disp('NFP\nmul');
  mul_Dot Product3_dotp_4 : Subsystem
      mask Display: disp('NFP\nmul');
  mul_Dot Product3_dotp_5 : Subsystem
      mask Display: disp('NFP\nmul');
  mul_Dot Product3_dotp_6 : Subsystem
      mask Display: disp('NFP\nmul');
  mul_Dot Product3_dotp_7 : Subsystem
      mask Display: disp('NFP\nmul');
  mul_Dot Product3_dotp_8 : Subsystem
      mask Display: disp('NFP\nmul');
  mul_Dot Product3_dotp_9 : Subsystem
      mask Display: disp('NFP\nmul');
  mul_Dot Product4_dotp_0 : Subsystem
      mask Display: disp('NFP\nmul');
  mul_Dot Product4_dotp_1 : Subsystem
      mask Display: disp('NFP\nmul');
  mul_Dot Product4_dotp_10 : Subsystem
      mask Display: disp('NFP\nmul');
  mul_Dot Product4_dotp_11 : Subsystem
      mask Display: disp('NFP\nmul');
  mul_Dot Product4_dotp_12 : Subsystem
      mask Display: disp('NFP\nmul');
  mul_Dot Product4_dotp_13 : Subsystem
      mask Display: disp('NFP\nmul');
  mul_Dot Product4_dotp_14 : Subsystem
      mask Display: disp('NFP\nmul');
  mul_Dot Product4_dotp_15 : Subsystem
      mask Display: disp('NFP\nmul');
  mul_Dot Product4_dotp_2 : Subsystem
      mask Display: disp('NFP\nmul');
  mul_Dot Product4_dotp_3 : Subsystem
      mask Display: disp('NFP\nmul');
  mul_Dot Product4_dotp_4 : Subsystem
      mask Display: disp('NFP\nmul');
  mul_Dot Product4_dotp_5 : Subsystem
      mask Display: disp('NFP\nmul');
  mul_Dot Product4_dotp_6 : Subsystem
      mask Display: disp('NFP\nmul');
  mul_Dot Product4_dotp_7 : Subsystem
      mask Display: disp('NFP\nmul');
  mul_Dot Product4_dotp_8 : Subsystem
      mask Display: disp('NFP\nmul');
  mul_Dot Product4_dotp_9 : Subsystem
      mask Display: disp('NFP\nmul');
  mul_Dot Product5_dotp_0 : Subsystem
      mask Display: disp('NFP\nmul');
  mul_Dot Product5_dotp_1 : Subsystem
      mask Display: disp('NFP\nmul');
  mul_Dot Product5_dotp_10 : Subsystem
      mask Display: disp('NFP\nmul');
  mul_Dot Product5_dotp_11 : Subsystem
      mask Display: disp('NFP\nmul');
  mul_Dot Product5_dotp_12 : Subsystem
      mask Display: disp('NFP\nmul');
  mul_Dot Product5_dotp_13 : Subsystem
      mask Display: disp('NFP\nmul');
  mul_Dot Product5_dotp_14 : Subsystem
      mask Display: disp('NFP\nmul');
  mul_Dot Product5_dotp_15 : Subsystem
      mask Display: disp('NFP\nmul');
  mul_Dot Product5_dotp_2 : Subsystem
      mask Display: disp('NFP\nmul');
  mul_Dot Product5_dotp_3 : Subsystem
      mask Display: disp('NFP\nmul');
  mul_Dot Product5_dotp_4 : Subsystem
      mask Display: disp('NFP\nmul');
  mul_Dot Product5_dotp_5 : Subsystem
      mask Display: disp('NFP\nmul');
  mul_Dot Product5_dotp_6 : Subsystem
      mask Display: disp('NFP\nmul');
  mul_Dot Product5_dotp_7 : Subsystem
      mask Display: disp('NFP\nmul');
  mul_Dot Product5_dotp_8 : Subsystem
      mask Display: disp('NFP\nmul');
  mul_Dot Product5_dotp_9 : Subsystem
      mask Display: disp('NFP\nmul');
  mul_Dot Product6_dotp_0 : Subsystem
      mask Display: disp('NFP\nmul');
  mul_Dot Product6_dotp_1 : Subsystem
      mask Display: disp('NFP\nmul');
  mul_Dot Product6_dotp_10 : Subsystem
      mask Display: disp('NFP\nmul');
  mul_Dot Product6_dotp_11 : Subsystem
      mask Display: disp('NFP\nmul');
  mul_Dot Product6_dotp_12 : Subsystem
      mask Display: disp('NFP\nmul');
  mul_Dot Product6_dotp_13 : Subsystem
      mask Display: disp('NFP\nmul');
  mul_Dot Product6_dotp_14 : Subsystem
      mask Display: disp('NFP\nmul');
  mul_Dot Product6_dotp_15 : Subsystem
      mask Display: disp('NFP\nmul');
  mul_Dot Product6_dotp_2 : Subsystem
      mask Display: disp('NFP\nmul');
  mul_Dot Product6_dotp_3 : Subsystem
      mask Display: disp('NFP\nmul');
  mul_Dot Product6_dotp_4 : Subsystem
      mask Display: disp('NFP\nmul');
  mul_Dot Product6_dotp_5 : Subsystem
      mask Display: disp('NFP\nmul');
  mul_Dot Product6_dotp_6 : Subsystem
      mask Display: disp('NFP\nmul');
  mul_Dot Product6_dotp_7 : Subsystem
      mask Display: disp('NFP\nmul');
  mul_Dot Product6_dotp_8 : Subsystem
      mask Display: disp('NFP\nmul');
  mul_Dot Product6_dotp_9 : Subsystem
      mask Display: disp('NFP\nmul');
  mul_Dot Product7_dotp_0 : Subsystem
      mask Display: disp('NFP\nmul');
  mul_Dot Product7_dotp_1 : Subsystem
      mask Display: disp('NFP\nmul');
  mul_Dot Product7_dotp_10 : Subsystem
      mask Display: disp('NFP\nmul');
  mul_Dot Product7_dotp_11 : Subsystem
      mask Display: disp('NFP\nmul');
  mul_Dot Product7_dotp_12 : Subsystem
      mask Display: disp('NFP\nmul');
  mul_Dot Product7_dotp_13 : Subsystem
      mask Display: disp('NFP\nmul');
  mul_Dot Product7_dotp_14 : Subsystem
      mask Display: disp('NFP\nmul');
  mul_Dot Product7_dotp_15 : Subsystem
      mask Display: disp('NFP\nmul');
  mul_Dot Product7_dotp_2 : Subsystem
      mask Display: disp('NFP\nmul');
  mul_Dot Product7_dotp_3 : Subsystem
      mask Display: disp('NFP\nmul');
  mul_Dot Product7_dotp_4 : Subsystem
      mask Display: disp('NFP\nmul');
  mul_Dot Product7_dotp_5 : Subsystem
      mask Display: disp('NFP\nmul');
  mul_Dot Product7_dotp_6 : Subsystem
      mask Display: disp('NFP\nmul');
  mul_Dot Product7_dotp_7 : Subsystem
      mask Display: disp('NFP\nmul');
  mul_Dot Product7_dotp_8 : Subsystem
      mask Display: disp('NFP\nmul');
  mul_Dot Product7_dotp_9 : Subsystem
      mask Display: disp('NFP\nmul');
  mul_Dot Product8_dotp_0 : Subsystem
      mask Display: disp('NFP\nmul');
  mul_Dot Product8_dotp_1 : Subsystem
      mask Display: disp('NFP\nmul');
  mul_Dot Product8_dotp_10 : Subsystem
      mask Display: disp('NFP\nmul');
  mul_Dot Product8_dotp_11 : Subsystem
      mask Display: disp('NFP\nmul');
  mul_Dot Product8_dotp_12 : Subsystem
      mask Display: disp('NFP\nmul');
  mul_Dot Product8_dotp_13 : Subsystem
      mask Display: disp('NFP\nmul');
  mul_Dot Product8_dotp_14 : Subsystem
      mask Display: disp('NFP\nmul');
  mul_Dot Product8_dotp_15 : Subsystem
      mask Display: disp('NFP\nmul');
  mul_Dot Product8_dotp_2 : Subsystem
      mask Display: disp('NFP\nmul');
  mul_Dot Product8_dotp_3 : Subsystem
      mask Display: disp('NFP\nmul');
  mul_Dot Product8_dotp_4 : Subsystem
      mask Display: disp('NFP\nmul');
  mul_Dot Product8_dotp_5 : Subsystem
      mask Display: disp('NFP\nmul');
  mul_Dot Product8_dotp_6 : Subsystem
      mask Display: disp('NFP\nmul');
  mul_Dot Product8_dotp_7 : Subsystem
      mask Display: disp('NFP\nmul');
  mul_Dot Product8_dotp_8 : Subsystem
      mask Display: disp('NFP\nmul');
  mul_Dot Product8_dotp_9 : Subsystem
      mask Display: disp('NFP\nmul');
  mul_Dot Product9_dotp_0 : Subsystem
      mask Display: disp('NFP\nmul');
  mul_Dot Product9_dotp_1 : Subsystem
      mask Display: disp('NFP\nmul');
  mul_Dot Product9_dotp_10 : Subsystem
      mask Display: disp('NFP\nmul');
  mul_Dot Product9_dotp_11 : Subsystem
      mask Display: disp('NFP\nmul');
  mul_Dot Product9_dotp_12 : Subsystem
      mask Display: disp('NFP\nmul');
  mul_Dot Product9_dotp_13 : Subsystem
      mask Display: disp('NFP\nmul');
  mul_Dot Product9_dotp_14 : Subsystem
      mask Display: disp('NFP\nmul');
  mul_Dot Product9_dotp_15 : Subsystem
      mask Display: disp('NFP\nmul');
  mul_Dot Product9_dotp_2 : Subsystem
      mask Display: disp('NFP\nmul');
  mul_Dot Product9_dotp_3 : Subsystem
      mask Display: disp('NFP\nmul');
  mul_Dot Product9_dotp_4 : Subsystem
      mask Display: disp('NFP\nmul');
  mul_Dot Product9_dotp_5 : Subsystem
      mask Display: disp('NFP\nmul');
  mul_Dot Product9_dotp_6 : Subsystem
      mask Display: disp('NFP\nmul');
  mul_Dot Product9_dotp_7 : Subsystem
      mask Display: disp('NFP\nmul');
  mul_Dot Product9_dotp_8 : Subsystem
      mask Display: disp('NFP\nmul');
  mul_Dot Product9_dotp_9 : Subsystem
      mask Display: disp('NFP\nmul');
  mul_Dot Product_dotp_0 : Subsystem
      mask Display: disp('NFP\nmul');
  mul_Dot Product_dotp_1 : Subsystem
      mask Display: disp('NFP\nmul');
  mul_Dot Product_dotp_10 : Subsystem
      mask Display: disp('NFP\nmul');
  mul_Dot Product_dotp_11 : Subsystem
      mask Display: disp('NFP\nmul');
  mul_Dot Product_dotp_12 : Subsystem
      mask Display: disp('NFP\nmul');
  mul_Dot Product_dotp_13 : Subsystem
      mask Display: disp('NFP\nmul');
  mul_Dot Product_dotp_14 : Subsystem
      mask Display: disp('NFP\nmul');
  mul_Dot Product_dotp_15 : Subsystem
      mask Display: disp('NFP\nmul');
  mul_Dot Product_dotp_2 : Subsystem
      mask Display: disp('NFP\nmul');
  mul_Dot Product_dotp_3 : Subsystem
      mask Display: disp('NFP\nmul');
  mul_Dot Product_dotp_4 : Subsystem
      mask Display: disp('NFP\nmul');
  mul_Dot Product_dotp_5 : Subsystem
      mask Display: disp('NFP\nmul');
  mul_Dot Product_dotp_6 : Subsystem
      mask Display: disp('NFP\nmul');
  mul_Dot Product_dotp_7 : Subsystem
      mask Display: disp('NFP\nmul');
  mul_Dot Product_dotp_8 : Subsystem
      mask Display: disp('NFP\nmul');
  mul_Dot Product_dotp_9 : Subsystem
      mask Display: disp('NFP\nmul');
  mux : Mux  Inputs=5
  mux1 : Mux  Inputs=16
  mux2 : Mux  Inputs=16
  t : RateTransition  InitialCondition=double(0)  OutPortSampleTimeOpt=Multiple of input port sample time  OutPortSampleTimeMultiple=166
  t1 : RateTransition  InitialCondition=double(0)  OutPortSampleTimeOpt=Multiple of input port sample time  OutPortSampleTimeMultiple=166
  t{3,6..37} (33 alike) : Demux  Outputs=16
  t2 : Demux  Outputs=3
  t38 : Constant  Value=fi(1,0,8,0)  OutDataTypeStr=uint8  SampleTime=6.02409638554217e-09
  t39 : Switch  Threshold=double(1)  OutDataTypeStr=uint8  SampleTime=6.02409638554217e-09  SaturateOnIntegerOverflow=off  InputSameDT=off
  t4 : Demux  Outputs=5
  t5 : Demux  Outputs=11
  user_out : Outport  SampleTime=1e-06
  user_out_clk : Outport  Port=2  SampleTime=1e-06
  user_out_8sig : Outport  Port=3  SampleTime=1e-06
  wires:
  t34/7 -> delayMatch443/1
  Dot Product12/1(Out1) -> Dot Product13/2(In2)
  delayMatch199/1 -> mul_Dot Product6_dotp_10/1(In1)
  Dot Product109/1(Out1) -> Dot Product1010/2(In2)
  t34/1 -> delayMatch449/1
  Index Vector_dtc_comp/1 -> delayMatch494/1
  t30/12 -> delayMatch378/1
  delayMatch405/1 -> mul_Dot Product13_dotp_14/1(In1)
  t24/13 -> delayMatch287/1
  t30/14 -> delayMatch376/1
  Dot Product78/1(Out1) -> Dot Product79/2(In2)
  mul_Dot Product1_dotp_9/1(Out1) -> delayMatch67/1
  t2/2 -> delayMatch1/1
  delayMatch427/1 -> Dot Product139/1(In1)
  t24/10 -> delayMatch290/1
  t34/4 -> delayMatch446/1
  Dot Product103/1(Out1) -> Dot Product104/2(In2)
  mul_Dot Product10_dotp_0/1(Out1) -> Dot Product101/2(In2)
  delayMatch84/1 -> mul_Dot Product2_dotp_5/1(In1)
  Dot Product1414/1(Out1) -> Dot Product1415/2(In2)
  Dot Product1122/1(Out1) -> Dot Product1123/2(In2)
  mul_Dot Product9_dotp_1/1(Out1) -> Dot Product91/1(In1)
  delayMatch454/1 -> Dot Product146/1(In1)
  t16/15 -> delayMatch165/1
  t37/1 -> mul_Dot Product15_dotp_0/2(In2)
  mul_Dot Product2_dotp_3/1(Out1) -> delayMatch91/1
  delayMatch297/1 -> mul_Dot Product9_dotp_2/1(In1)
  t3/5 -> Demux_mux_1/5
  mul_Dot Product10_dotp_6/1(Out1) -> delayMatch334/1
  delayMatch239/1 -> mul_Dot Product7_dotp_0/1(In1)
  Dot Product95/1(Out1) -> Dot Product96/2(In2)
  delayMatch154/1 -> Dot Product46/1(In1)
  delayMatch/1 -> mux/3
  t20/2 -> delayMatch238/1
  t3/10 -> Mux4_out1_9_term9/1
  Data Type Conversion2/1 -> mux/2
  Dot Product411/1(Out1) -> Dot Product412/2(In2)
  delayMatch381/1 -> mul_Dot Product12_dotp_8/1(In1)
  t19/16 -> mul_Dot Product6_dotp_15/2(In2)
  Dot Product212/1(Out1) -> Dot Product213/2(In2)
  delayMatch477/1 -> mul_Dot Product15_dotp_2/1(In1)
  delayMatch479/1 -> mul_Dot Product15_dotp_0/1(In1)
  delayMatch296/1 -> mul_Dot Product9_dotp_3/1(In1)
  Selector13/1 -> t32/1
  Dot Product79/1(Out1) -> Dot Product710/2(In2)
  t15/1 -> mul_Dot Product4_dotp_0/2(In2)
  mul_Dot Product8_dotp_8/1(Out1) -> delayMatch276/1
  mul_Dot Product4_dotp_5/1(Out1) -> delayMatch153/1
  t35/8 -> mul_Dot Product14_dotp_7/2(In2)
  Dot Product132/1(Out1) -> Dot Product133/2(In2)
  t39/1 -> Selector16/2
  mul_Dot Product14_dotp_10/1(Out1) -> delayMatch458/1
  t34/14 -> delayMatch436/1
  delayMatch228/1 -> mul_Dot Product7_dotp_11/1(In1)
  t34/10 -> delayMatch440/1
  delayMatch33/1 -> Dot Product4/1(In1)
  t6/3 -> delayMatch27/1
  delayMatch227/1 -> mul_Dot Product7_dotp_12/1(In1)
  t24/3 -> delayMatch297/1
  t34/13 -> delayMatch437/1
  mul_Dot Product5_dotp_6/1(Out1) -> delayMatch184/1
  mul_Dot Product3_dotp_3/1(Out1) -> delayMatch121/1
  mul_Dot Product2_dotp_1/1(Out1) -> Dot Product21/1(In1)
  Dot Product135/1(Out1) -> Dot Product136/2(In2)
  Dot Product1113/1(Out1) -> Dot Product1114/2(In2)
  t14/13 -> delayMatch137/1
  delayMatch32/1 -> Dot Product3/1(In1)
  t35/15 -> mul_Dot Product14_dotp_14/2(In2)
  mul_Dot Product14_dotp_4/1(Out1) -> delayMatch452/1
  delayMatch142/1 -> mul_Dot Product4_dotp_7/1(In1)
  Dot Product125/1(Out1) -> Dot Product126/2(In2)
  delayMatch278/1 -> Dot Product810/1(In1)
  t20/13 -> delayMatch227/1
  t24/2 -> delayMatch298/1
  t17/14 -> mul_Dot Product5_dotp_13/2(In2)
  t36/2 -> delayMatch478/1
  t22/5 -> delayMatch265/1
  t33/1 -> mul_Dot Product13_dotp_0/2(In2)
  t26/8 -> delayMatch322/1
  t18/16 -> delayMatch194/1
  t26/14 -> delayMatch316/1
  mul_Dot Product13_dotp_14/1(Out1) -> delayMatch432/1
  delayMatch424/1 -> Dot Product136/1(In1)
  Dot Product15/1(Out1) -> Dot Product16/2(In2)
  Dot Product611/1(Out1) -> Dot Product612/2(In2)
  Dot Product415/1(Out1) -> mux1/5
  t15/13 -> mul_Dot Product4_dotp_12/2(In2)
  mul_Dot Product11_dotp_2/1(Out1) -> delayMatch360/1
  delayMatch166/1 -> mul_Dot Product5_dotp_13/1(In1)
  t17/2 -> mul_Dot Product5_dotp_1/2(In2)
  PWM Generator/2(glo) -> Data Type Conversion2/1
  t21/7 -> mul_Dot Product7_dotp_6/2(In2)
  Dot Product41/1(Out1) -> Dot Product42/2(In2)
  delayMatch2/1 -> mux/5
  mul_Dot Product12_dotp_2/1(Out1) -> delayMatch390/1
  t30/5 -> delayMatch385/1
  t22/7 -> delayMatch263/1
  t16/3 -> delayMatch177/1
  delayMatch74/1 -> mul_Dot Product2_dotp_15/1(In1)
  mul_Dot Product4_dotp_14/1(Out1) -> delayMatch162/1
  mul_Dot Product2_dotp_11/1(Out1) -> delayMatch99/1
  t5/10 -> delayMatch12/1
  t37/5 -> mul_Dot Product15_dotp_4/2(In2)
  delayMatch281/1 -> Dot Product813/1(In1)
  t21/8 -> mul_Dot Product7_dotp_7/2(In2)
  t15/4 -> mul_Dot Product4_dotp_3/2(In2)
  mul_Dot Product14_dotp_0/1(Out1) -> Dot Product141/2(In2)
  t26/7 -> delayMatch323/1
  delayMatch331/1 -> Dot Product103/1(In1)
  delayMatch124/1 -> Dot Product36/1(In1)
  delayMatch418/1 -> mul_Dot Product13_dotp_1/1(In1)
  mul_Dot Product_dotp_5/1(Out1) -> delayMatch33/1
  t22/8 -> delayMatch262/1
  t26/5 -> delayMatch325/1
  t32/6 -> delayMatch414/1
  t32/4 -> delayMatch416/1
  mul_Dot Product5_dotp_10/1(Out1) -> delayMatch188/1
  delayMatch416/1 -> mul_Dot Product13_dotp_3/1(In1)
  t12/8 -> delayMatch112/1
  Dot Product1215/1(Out1) -> mux1/13
  delayMatch4/1 -> mux2/7
  t35/3 -> mul_Dot Product14_dotp_2/2(In2)
  t3/12 -> Mux4_out1_11_term11/1
  Dot Product92/1(Out1) -> Dot Product93/2(In2)
  t13/9 -> mul_Dot Product3_dotp_8/2(In2)
  t16/8 -> delayMatch172/1
  t22/14 -> delayMatch256/1
  delayMatch22/1 -> mul_Dot Product_dotp_7/1(In1)
  t25/12 -> mul_Dot Product9_dotp_11/2(In2)
  t9/8 -> mul_Dot Product1_dotp_7/2(In2)
  t33/3 -> mul_Dot Product13_dotp_2/2(In2)
  Dot Product912/1(Out1) -> Dot Product913/2(In2)
  Dot Product139/1(Out1) -> Dot Product1310/2(In2)
  t13/8 -> mul_Dot Product3_dotp_7/2(In2)
  t27/1 -> mul_Dot Product10_dotp_0/2(In2)
  t34/16 -> delayMatch434/1
  t19/13 -> mul_Dot Product6_dotp_12/2(In2)
  Dot Product1511/1(Out1) -> Dot Product1512/2(In2)
  t10/9 -> delayMatch81/1
  t30/11 -> delayMatch379/1
  Dot Product149/1(Out1) -> Dot Product1410/2(In2)
  Dot Product159/1(Out1) -> Dot Product1510/2(In2)
  mul_Dot Product_dotp_12/1(Out1) -> delayMatch40/1
  t2/1 -> delayMatch/1
  t30/13 -> delayMatch377/1
  delayMatch219/1 -> Dot Product611/1(In1)
  t2/3 -> delayMatch2/1
  t28/9 -> delayMatch351/1
  Dot Product154/1(Out1) -> Dot Product155/2(In2)
  Index Vector/1 -> t/1
  Dot Product612/1(Out1) -> Dot Product613/2(In2)
  t38/1 -> t39/3
  mul_Dot Product12_dotp_4/1(Out1) -> delayMatch392/1
  delayMatch453/1 -> Dot Product145/1(In1)
  Dot Product116/1(Out1) -> Dot Product117/2(In2)
  delayMatch357/1 -> mul_Dot Product11_dotp_2/1(In1)
  t16/14 -> delayMatch166/1
  t36/16 -> delayMatch464/1
  t10/11 -> delayMatch79/1
  t16/16 -> delayMatch164/1
  delayMatch455/1 -> Dot Product147/1(In1)
  delayMatch272/1 -> Dot Product84/1(In1)
  t23/15 -> mul_Dot Product8_dotp_14/2(In2)
  t9/14 -> mul_Dot Product1_dotp_13/2(In2)
  t31/12 -> mul_Dot Product12_dotp_11/2(In2)
  t25/15 -> mul_Dot Product9_dotp_14/2(In2)
  mul_Dot Product8_dotp_5/1(Out1) -> delayMatch273/1
  Dot Product134/1(Out1) -> Dot Product135/2(In2)
  delayMatch1/1 -> mux/4
  t8/6 -> delayMatch54/1
  t30/4 -> delayMatch386/1
  Dot Product913/1(Out1) -> Dot Product914/2(In2)
  t5/3 -> delayMatch5/1
  Data Type Conversion1/1 -> mux/1
  Dot Product136/1(Out1) -> Dot Product137/2(In2)
  t36/3 -> delayMatch477/1
  t6/2 -> delayMatch28/1
  t36/1 -> delayMatch479/1
  Dot Product156/1(Out1) -> Dot Product157/2(In2)
  delayMatch263/1 -> mul_Dot Product8_dotp_6/1(In1)
  Dot Product1412/1(Out1) -> Dot Product1413/2(In2)
  Dot Product711/1(Out1) -> Dot Product712/2(In2)
  delayMatch98/1 -> Dot Product210/1(In1)
  t20/10 -> delayMatch230/1
  t36/7 -> delayMatch473/1
  t10/5 -> delayMatch85/1
  t36/4 -> delayMatch476/1
  delayMatch10/1 -> mux2/13
  delayMatch208/1 -> mul_Dot Product6_dotp_1/1(In1)
  t32/7 -> delayMatch413/1
  mul_Dot Product4_dotp_2/1(Out1) -> delayMatch150/1
  delayMatch461/1 -> Dot Product1413/1(In1)
  Selector16/1 -> t1/1
  delayMatch489/1 -> Dot Product1511/1(In1)
  delayMatch96/1 -> Dot Product28/1(In1)
  mul_Dot Product12_dotp_10/1(Out1) -> delayMatch398/1
  delayMatch330/1 -> Dot Product102/1(In1)
  t18/5 -> delayMatch205/1
  t36/5 -> delayMatch475/1
  Dot Product1411/1(Out1) -> Dot Product1412/2(In2)
  t15/11 -> mul_Dot Product4_dotp_10/2(In2)
  Dot Product61/1(Out1) -> Dot Product62/2(In2)
  Dot Product105/1(Out1) -> Dot Product106/2(In2)
  Dot Product102/1(Out1) -> Dot Product103/2(In2)
  t12/9 -> delayMatch111/1
  t8/4 -> delayMatch56/1
  delayMatch161/1 -> Dot Product413/1(In1)
  delayMatch246/1 -> Dot Product78/1(In1)
  Dot Product915/1(Out1) -> mux1/10
  t19/4 -> mul_Dot Product6_dotp_3/2(In2)
  t12/13 -> delayMatch107/1
  t32/15 -> delayMatch405/1
  t26/12 -> delayMatch318/1
  t10/10 -> delayMatch80/1
  Dot Product1118/1(Out1) -> Dot Product1119/2(In2)
  delayMatch104/1 -> mul_Dot Product3_dotp_15/1(In1)
  delayMatch430/1 -> Dot Product1312/1(In1)
  delayMatch58/1 -> mul_Dot Product1_dotp_1/1(In1)
  Dot Product1111/1(Out1) -> Dot Product1112/2(In2)
  Dot Product1415/1(Out1) -> mux1/15
  delayMatch411/1 -> mul_Dot Product13_dotp_8/1(In1)
  delayMatch207/1 -> mul_Dot Product6_dotp_2/1(In1)
  t6/8 -> delayMatch22/1
  t36/6 -> delayMatch474/1
  t3/16 -> Mux4_out1_15_term15/1
  t34/6 -> delayMatch444/1
  delayMatch342/1 -> Dot Product1014/1(In1)
  t24/8 -> delayMatch292/1
  t36/8 -> delayMatch472/1
  delayMatch490/1 -> Dot Product1512/1(In1)
  Dot Product22/1(Out1) -> Dot Product23/2(In2)
  t36/9 -> delayMatch471/1
  t8/3 -> delayMatch57/1
  delayMatch348/1 -> mul_Dot Product11_dotp_11/1(In1)
  t29/1 -> mul_Dot Product11_dotp_0/2(In2)
  delayMatch12/1 -> mux2/15
  t36/10 -> delayMatch470/1
  delayMatch120/1 -> Dot Product32/1(In1)
  delayMatch414/1 -> mul_Dot Product13_dotp_5/1(In1)
  mul_Dot Product11_dotp_6/1(Out1) -> delayMatch364/1
  t18/4 -> delayMatch206/1
  t18/3 -> delayMatch207/1
  t36/11 -> delayMatch469/1
  mul_Dot Product8_dotp_0/1(Out1) -> Dot Product81/2(In2)
  t6/15 -> delayMatch15/1
  Dot Product31/1(Out1) -> Dot Product32/2(In2)
  delayMatch328/1 -> mul_Dot Product10_dotp_1/1(In1)
  t31/9 -> mul_Dot Product12_dotp_8/2(In2)
  t14/12 -> delayMatch138/1
  t9/11 -> mul_Dot Product1_dotp_10/2(In2)
  mul_Dot Product11_dotp_11/1(Out1) -> delayMatch369/1
  t37/7 -> mul_Dot Product15_dotp_6/2(In2)
  delayMatch442/1 -> mul_Dot Product14_dotp_7/1(In1)
  delayMatch170/1 -> mul_Dot Product5_dotp_9/1(In1)
  mul_Dot Product13_dotp_1/1(Out1) -> Dot Product131/1(In1)
  Dot Product93/1(Out1) -> Dot Product94/2(In2)
  Dot Product54/1(Out1) -> Dot Product55/2(In2)
  delayMatch354/1 -> mul_Dot Product11_dotp_5/1(In1)
  delayMatch188/1 -> Dot Product510/1(In1)
  mul_Dot Product6_dotp_4/1(Out1) -> delayMatch212/1
  t18/1 -> delayMatch209/1
  t20/8 -> delayMatch232/1
  t14/3 -> delayMatch147/1
  Dot Product18/1(Out1) -> Dot Product19/2(In2)
  t28/2 -> delayMatch358/1
  t32/1 -> delayMatch419/1
  t34/11 -> delayMatch439/1
  t14/9 -> delayMatch141/1
  delayMatch307/1 -> Dot Product99/1(In1)
  Dot Product48/1(Out1) -> Dot Product49/2(In2)
  mul_Dot Product13_dotp_3/1(Out1) -> delayMatch421/1
  t25/10 -> mul_Dot Product9_dotp_9/2(In2)
  Dot Product83/1(Out1) -> Dot Product84/2(In2)
  t33/9 -> mul_Dot Product13_dotp_8/2(In2)
  delayMatch368/1 -> Dot Product1119/1(In1)
  delayMatch274/1 -> Dot Product86/1(In1)
  delayMatch268/1 -> mul_Dot Product8_dotp_1/1(In1)
  t10/13 -> delayMatch77/1
  t36/12 -> delayMatch468/1
  mul_Dot Product1_dotp_3/1(Out1) -> delayMatch61/1
  t26/10 -> delayMatch320/1
  t32/13 -> delayMatch407/1
  mux2/1 -> t9/1, t7/1, t11/1, t15/1, t21/1, t23/1, t37/1, t27/1, t25/1, t13/1, t35/1, t31/1, t33/1, t17/1, t29/1, t19/1
  mul_Dot Product6_dotp_1/1(Out1) -> Dot Product61/1(In1)
  Dot Product1124/1(Out1) -> mux1/12
  t8/14 -> delayMatch46/1
  t28/16 -> delayMatch344/1
  Dot Product46/1(Out1) -> Dot Product47/2(In2)
  t17/7 -> mul_Dot Product5_dotp_6/2(In2)
  t21/2 -> mul_Dot Product7_dotp_1/2(In2)
  delayMatch17/1 -> mul_Dot Product_dotp_12/1(In1)
  mul_Dot Product5_dotp_8/1(Out1) -> delayMatch186/1
  t6/6 -> delayMatch24/1
  t10/12 -> delayMatch78/1
  t36/15 -> delayMatch465/1
  Dot Product38/1(Out1) -> Dot Product39/2(In2)
  t16/1 -> delayMatch179/1
  t37/11 -> mul_Dot Product15_dotp_10/2(In2)
  t36/13 -> delayMatch467/1
  Dot Product147/1(Out1) -> Dot Product148/2(In2)
  Dot Product410/1(Out1) -> Dot Product411/2(In2)
  t16/12 -> delayMatch168/1
  t36/14 -> delayMatch466/1
  t6/5 -> delayMatch25/1
  delayMatch483/1 -> Dot Product155/1(In1)
  Dot Product42/1(Out1) -> Dot Product43/2(In2)
  t34/2 -> delayMatch448/1
  delayMatch349/1 -> mul_Dot Product11_dotp_10/1(In1)
  Dot Product128/1(Out1) -> Dot Product129/2(In2)
  t11/16 -> mul_Dot Product2_dotp_15/2(In2)
  t8/15 -> delayMatch45/1
  t23/4 -> mul_Dot Product8_dotp_3/2(In2)
  t33/14 -> mul_Dot Product13_dotp_13/2(In2)
  mul_Dot Product12_dotp_0/1(Out1) -> Dot Product121/2(In2)
  mul_Dot Product10_dotp_7/1(Out1) -> delayMatch335/1
  delayMatch474/1 -> mul_Dot Product15_dotp_5/1(In1)
  t10/4 -> delayMatch86/1
  t34/3 -> delayMatch447/1
  mul_Dot Product7_dotp_14/1(Out1) -> delayMatch252/1
  Dot Product1119/1(Out1) -> Dot Product1120/2(In2)
  Dot Product613/1(Out1) -> Dot Product614/2(In2)
  t14/14 -> delayMatch136/1
  t34/8 -> delayMatch442/1
  t7/16 -> mul_Dot Product_dotp_15/2(In2)
  t12/15 -> delayMatch105/1
  mul_Dot Product11_dotp_4/1(Out1) -> delayMatch362/1
  t15/15 -> mul_Dot Product4_dotp_14/2(In2)
  t29/14 -> mul_Dot Product11_dotp_13/2(In2)
  delayMatch35/1 -> Dot Product6/1(In1)
  mul_Dot Product13_dotp_2/1(Out1) -> delayMatch420/1
  t24/11 -> delayMatch289/1
  t34/5 -> delayMatch445/1
  Dot Product99/1(Out1) -> Dot Product910/2(In2)
  t20/9 -> delayMatch231/1
  t14/2 -> delayMatch148/1
  delayMatch97/1 -> Dot Product29/1(In1)
  delayMatch488/1 -> Dot Product1510/1(In1)
  delayMatch91/1 -> Dot Product23/1(In1)
  Delay_Switch/1 -> Unit Delay Enabled Synchronous22_lowered/1
  Dot Product17/1(Out1) -> Dot Product18/2(In2)
  Dot Product82/1(Out1) -> Dot Product83/2(In2)
  mul_Dot Product5_dotp_3/1(Out1) -> delayMatch181/1
  t8/9 -> delayMatch51/1
  t12/4 -> delayMatch116/1
  delayMatch93/1 -> Dot Product25/1(In1)
  t26/6 -> delayMatch324/1
  t6/4 -> delayMatch26/1
  delayMatch358/1 -> mul_Dot Product11_dotp_1/1(In1)
  t16/13 -> delayMatch167/1
  t20/6 -> delayMatch234/1
  t14/1 -> delayMatch149/1
  delayMatch34/1 -> Dot Product5/1(In1)
  t6/7 -> delayMatch23/1
  t34/9 -> delayMatch441/1
  mul_Dot Product8_dotp_2/1(Out1) -> delayMatch270/1
  t34/12 -> delayMatch438/1
  t11/8 -> mul_Dot Product2_dotp_7/2(In2)
  t33/6 -> mul_Dot Product13_dotp_5/2(In2)
  delayMatch258/1 -> mul_Dot Product8_dotp_11/1(In1)
  Dot Product1014/1(Out1) -> Dot Product1015/2(In2)
  Dot Product10/1(Out1) -> Dot Product11/2(In2)
  delayMatch392/1 -> Dot Product124/1(In1)
  t34/15 -> delayMatch435/1
  delayMatch487/1 -> Dot Product159/1(In1)
  t16/6 -> delayMatch174/1
  t18/11 -> delayMatch199/1
  mul_Dot Product5_dotp_2/1(Out1) -> delayMatch180/1
  t24/5 -> delayMatch295/1
  t32/2 -> delayMatch418/1
  t24/4 -> delayMatch296/1
  t32/3 -> delayMatch417/1
  mul_Dot Product5_dotp_7/1(Out1) -> delayMatch185/1
  t12/11 -> delayMatch109/1
  delayMatch332/1 -> Dot Product104/1(In1)
  delayMatch8/1 -> mux2/11
  t22/11 -> delayMatch259/1
  t32/5 -> delayMatch415/1
  t8/5 -> delayMatch55/1
  t30/3 -> delayMatch387/1
  mul_Dot Product5_dotp_1/1(Out1) -> Dot Product51/1(In1)
  t32/8 -> delayMatch412/1
  Dot Product514/1(Out1) -> Dot Product515/2(In2)
  t28/14 -> delayMatch346/1
  Dot Product1112/1(Out1) -> Dot Product1113/2(In2)
  Dot Product121/1(Out1) -> Dot Product122/2(In2)
  Dot Product412/1(Out1) -> Dot Product413/2(In2)
  Dot Product29/1(Out1) -> Dot Product210/2(In2)
  t22/15 -> delayMatch255/1
  t32/9 -> delayMatch411/1
  Dot Product1514/1(Out1) -> Dot Product1515/2(In2)
  delayMatch355/1 -> mul_Dot Product11_dotp_4/1(In1)
  t19/7 -> mul_Dot Product6_dotp_6/2(In2)
  delayMatch312/1 -> Dot Product914/1(In1)
  delayMatch299/1 -> mul_Dot Product9_dotp_0/1(In1)
  delayMatch55/1 -> mul_Dot Product1_dotp_4/1(In1)
  t25/5 -> mul_Dot Product9_dotp_4/2(In2)
  t30/16 -> delayMatch374/1
  delayMatch447/1 -> mul_Dot Product14_dotp_2/1(In1)
  t4/5 -> mux2/5
  Delay/1 -> Delay_absorbed/1
  Dot Product71/1(Out1) -> Dot Product72/2(In2)
  t32/10 -> delayMatch410/1
  Dot Product55/1(Out1) -> Dot Product56/2(In2)
  t32/11 -> delayMatch409/1
  Dot Product414/1(Out1) -> Dot Product415/2(In2)
  t26/13 -> delayMatch317/1
  t32/14 -> delayMatch406/1
  delayMatch340/1 -> Dot Product1012/1(In1)
  Dot Product215/1(Out1) -> mux1/3
  delayMatch425/1 -> Dot Product137/1(In1)
  Dot Product510/1(Out1) -> Dot Product511/2(In2)
  delayMatch111/1 -> mul_Dot Product3_dotp_8/1(In1)
  t26/11 -> delayMatch319/1
  t32/12 -> delayMatch408/1
  t18/9 -> delayMatch201/1
  mul_Dot Product3_dotp_0/1(Out1) -> Dot Product31/2(In2)
  Dot Product1513/1(Out1) -> Dot Product1514/2(In2)
  Dot Product112/1(Out1) -> Dot Product113/2(In2)
  delayMatch179/1 -> mul_Dot Product5_dotp_0/1(In1)
  Dot Product1413/1(Out1) -> Dot Product1414/2(In2)
  mul_Dot Product8_dotp_1/1(Out1) -> Dot Product81/1(In1)
  delayMatch362/1 -> Dot Product1113/1(In1)
  delayMatch456/1 -> Dot Product148/1(In1)
  t16/9 -> delayMatch171/1
  delayMatch133/1 -> Dot Product315/1(In1)
  mul_Dot Product15_dotp_11/1(Out1) -> delayMatch489/1
  t25/1 -> mul_Dot Product9_dotp_0/2(In2)
  t12/14 -> delayMatch106/1
  t32/16 -> delayMatch404/1
  t12/10 -> delayMatch110/1
  t22/10 -> delayMatch260/1
  t30/1 -> delayMatch389/1
  mul_Dot Product9_dotp_15/1(Out1) -> delayMatch313/1
  mul_Dot Product7_dotp_9/1(Out1) -> delayMatch247/1
  t7/6 -> mul_Dot Product_dotp_5/2(In2)
  t30/2 -> delayMatch388/1
  t12/5 -> delayMatch115/1
  t8/8 -> delayMatch52/1
  t22/9 -> delayMatch261/1
  t30/6 -> delayMatch384/1
  Dot Product1120/1(Out1) -> Dot Product1121/2(In2)
  t17/8 -> mul_Dot Product5_dotp_7/2(In2)
  Dot Product106/1(Out1) -> Dot Product107/2(In2)
  mul_Dot Product10_dotp_15/1(Out1) -> delayMatch343/1
  t7/12 -> mul_Dot Product_dotp_11/2(In2)
  t30/7 -> delayMatch383/1
  delayMatch320/1 -> mul_Dot Product10_dotp_9/1(In1)
  t24/15 -> delayMatch285/1
  t30/8 -> delayMatch382/1
  t24/14 -> delayMatch286/1
  t30/9 -> delayMatch381/1
  delayMatch321/1 -> mul_Dot Product10_dotp_8/1(In1)
  Dot Product5/1(Out1) -> Dot Product6/2(In2)
  t22/2 -> delayMatch268/1
  t29/11 -> mul_Dot Product11_dotp_10/2(In2)
  t30/10 -> delayMatch380/1
  Dot Product153/1(Out1) -> Dot Product154/2(In2)
  mul_Dot Product14_dotp_2/1(Out1) -> delayMatch450/1
  t13/11 -> mul_Dot Product3_dotp_10/2(In2)
  t35/9 -> mul_Dot Product14_dotp_8/2(In2)
  mul_Dot Product7_dotp_2/1(Out1) -> delayMatch240/1
  mul_Dot Product4_dotp_6/1(Out1) -> delayMatch154/1
  Dot Product86/1(Out1) -> Dot Product87/2(In2)
  delayMatch92/1 -> Dot Product24/1(In1)
  delayMatch30/1 -> Dot Product1/1(In1)
  delayMatch230/1 -> mul_Dot Product7_dotp_9/1(In1)
  delayMatch145/1 -> mul_Dot Product4_dotp_4/1(In1)
  t10/3 -> delayMatch87/1
  t17/16 -> mul_Dot Product5_dotp_15/2(In2)
  mul_Dot Product15_dotp_0/1(Out1) -> Dot Product151/2(In2)
  Dot Product146/1(Out1) -> Dot Product147/2(In2)
  delayMatch468/1 -> mul_Dot Product15_dotp_11/1(In1)
  t20/12 -> delayMatch228/1
  t18/10 -> delayMatch200/1
  t16/7 -> delayMatch173/1
  Dot Product6/1(Out1) -> Dot Product7/2(In2)
  t24/12 -> delayMatch288/1
  t30/15 -> delayMatch375/1
  delayMatch46/1 -> mul_Dot Product1_dotp_13/1(In1)
  t28/1 -> delayMatch359/1
  delayMatch415/1 -> mul_Dot Product13_dotp_4/1(In1)
  delayMatch121/1 -> Dot Product33/1(In1)
  delayMatch206/1 -> mul_Dot Product6_dotp_3/1(In1)
  mul_Dot Product1_dotp_12/1(Out1) -> delayMatch70/1
  t24/9 -> delayMatch291/1
  t8/12 -> delayMatch48/1
  delayMatch48/1 -> mul_Dot Product1_dotp_11/1(In1)
  t28/3 -> delayMatch357/1
  Dot Product148/1(Out1) -> Dot Product149/2(In2)
  mul_Dot Product10_dotp_2/1(Out1) -> delayMatch330/1
  delayMatch463/1 -> Dot Product1415/1(In1)
  t28/4 -> delayMatch356/1
  Dot Product72/1(Out1) -> Dot Product73/2(In2)
  Dot Product67/1(Out1) -> Dot Product68/2(In2)
  mul_Dot Product_dotp_2/1(Out1) -> delayMatch30/1
  t3/11 -> Mux4_out1_10_term10/1
  delayMatch478/1 -> mul_Dot Product15_dotp_1/1(In1)
  delayMatch108/1 -> mul_Dot Product3_dotp_11/1(In1)
  Dot Product211/1(Out1) -> Dot Product212/2(In2)
  t29/12 -> mul_Dot Product11_dotp_11/2(In2)
  delayMatch434/1 -> mul_Dot Product14_dotp_15/1(In1)
  delayMatch101/1 -> Dot Product213/1(In1)
  t5/11 -> delayMatch13/1
  t5/6 -> delayMatch8/1
  delayMatch106/1 -> mul_Dot Product3_dotp_13/1(In1)
  delayMatch82/1 -> mul_Dot Product2_dotp_7/1(In1)
  t28/5 -> delayMatch355/1
  delayMatch81/1 -> mul_Dot Product2_dotp_8/1(In1)
  t28/6 -> delayMatch354/1
  mul_Dot Product9_dotp_2/1(Out1) -> delayMatch300/1
  Dot Product66/1(Out1) -> Dot Product67/2(In2)
  mul_Dot Product_dotp_6/1(Out1) -> delayMatch34/1
  delayMatch388/1 -> mul_Dot Product12_dotp_1/1(In1)
  Dot Product1310/1(Out1) -> Dot Product1311/2(In2)
  t28/7 -> delayMatch353/1
  delayMatch54/1 -> mul_Dot Product1_dotp_5/1(In1)
  Dot Product812/1(Out1) -> Dot Product813/2(In2)
  t17/13 -> mul_Dot Product5_dotp_12/2(In2)
  delayMatch234/1 -> mul_Dot Product7_dotp_5/1(In1)
  t20/14 -> delayMatch226/1
  t28/8 -> delayMatch352/1
  delayMatch302/1 -> Dot Product94/1(In1)
  delayMatch232/1 -> mul_Dot Product7_dotp_7/1(In1)
  t28/10 -> delayMatch350/1
  Dot Product39/1(Out1) -> Dot Product310/2(In2)
  mul_Dot Product10_dotp_14/1(Out1) -> delayMatch342/1
  delayMatch462/1 -> Dot Product1414/1(In1)
  t28/11 -> delayMatch349/1
  delayMatch378/1 -> mul_Dot Product12_dotp_11/1(In1)
  delayMatch472/1 -> mul_Dot Product15_dotp_7/1(In1)
  t22/16 -> delayMatch254/1
  t33/12 -> mul_Dot Product13_dotp_11/2(In2)
  delayMatch49/1 -> mul_Dot Product1_dotp_10/1(In1)
  Selector3/1 -> t12/1
  Dot Product33/1(Out1) -> Dot Product34/2(In2)
  t8/7 -> delayMatch53/1
  delayMatch70/1 -> Dot Product116/1(In1)
  t28/12 -> delayMatch348/1
  t23/1 -> mul_Dot Product8_dotp_0/2(In2)
  t9/2 -> mul_Dot Product1_dotp_1/2(In2)
  t11/11 -> mul_Dot Product2_dotp_10/2(In2)
  delayMatch157/1 -> Dot Product49/1(In1)
  Dot Product110/1(Out1) -> Dot Product111/2(In2)
  t12/3 -> delayMatch117/1
  delayMatch292/1 -> mul_Dot Product9_dotp_7/1(In1)
  t31/11 -> mul_Dot Product12_dotp_10/2(In2)
  t12/2 -> delayMatch118/1
  t28/13 -> delayMatch347/1
  mul_Dot Product6_dotp_7/1(Out1) -> delayMatch215/1
  t13/6 -> mul_Dot Product3_dotp_5/2(In2)
  t35/4 -> mul_Dot Product14_dotp_3/2(In2)
  mul_Dot Product4_dotp_7/1(Out1) -> delayMatch155/1
  mul_Dot Product13_dotp_7/1(Out1) -> delayMatch425/1
  delayMatch248/1 -> Dot Product710/1(In1)
  delayMatch286/1 -> mul_Dot Product9_dotp_13/1(In1)
  t16/2 -> delayMatch178/1
  t5/8 -> delayMatch10/1
  delayMatch377/1 -> mul_Dot Product12_dotp_12/1(In1)
  t23/3 -> mul_Dot Product8_dotp_2/2(In2)
  delayMatch159/1 -> Dot Product411/1(In1)
  t23/2 -> mul_Dot Product8_dotp_1/2(In2)
  t8/13 -> delayMatch47/1
  t26/1 -> delayMatch329/1
  t28/15 -> delayMatch345/1
  t26/16 -> delayMatch314/1
  t35/5 -> mul_Dot Product14_dotp_4/2(In2)
  Dot Product1012/1(Out1) -> Dot Product1013/2(In2)
  t26/2 -> delayMatch328/1
  t26/3 -> delayMatch327/1
  t26/4 -> delayMatch326/1
  Selector1/1 -> t8/1
  delayMatch406/1 -> mul_Dot Product13_dotp_13/1(In1)
  t13/12 -> mul_Dot Product3_dotp_11/2(In2)
  t19/6 -> mul_Dot Product6_dotp_5/2(In2)
  t11/9 -> mul_Dot Product2_dotp_8/2(In2)
  delayMatch444/1 -> mul_Dot Product14_dotp_5/1(In1)
  t26/9 -> delayMatch321/1
  Dot Product1410/1(Out1) -> Dot Product1411/2(In2)
  delayMatch137/1 -> mul_Dot Product4_dotp_12/1(In1)
  delayMatch222/1 -> Dot Product614/1(In1)
  Dot Product115/1(Out1) -> Dot Product116/2(In2)
  Selector9/1 -> t24/1
  delayMatch399/1 -> Dot Product1211/1(In1)
  mul_Dot Product1_dotp_2/1(Out1) -> delayMatch60/1
  delayMatch43/1 -> Dot Product14/1(In1)
  t26/15 -> delayMatch315/1
  Dot Product127/1(Out1) -> Dot Product128/2(In2)
  delayMatch469/1 -> mul_Dot Product15_dotp_10/1(In1)
  delayMatch481/1 -> Dot Product153/1(In1)
  mux1/1 -> Selector16/1, t3/1, Index Vector/2
  t24/1 -> delayMatch299/1
  delayMatch62/1 -> Dot Product18/1(In1)
  t14/15 -> delayMatch135/1
  mul_Dot Product7_dotp_11/1(Out1) -> delayMatch249/1
  mul_Dot Product2_dotp_7/1(Out1) -> delayMatch95/1
  delayMatch391/1 -> Dot Product123/1(In1)
  t19/11 -> mul_Dot Product6_dotp_10/2(In2)
  mul_Dot Product2_dotp_0/1(Out1) -> Dot Product21/2(In2)
  t18/8 -> delayMatch202/1
  delayMatch57/1 -> mul_Dot Product1_dotp_2/1(In1)
  delayMatch215/1 -> Dot Product67/1(In1)
  t14/6 -> delayMatch144/1
  t24/6 -> delayMatch294/1
  t10/6 -> delayMatch84/1
  t24/7 -> delayMatch293/1
  mul_Dot Product10_dotp_12/1(Out1) -> delayMatch340/1
  mux/1 -> LC vectorized/1(gate)
  t18/14 -> delayMatch196/1
  delayMatch486/1 -> Dot Product158/1(In1)
  mul_Dot Product3_dotp_9/1(Out1) -> delayMatch127/1
  delayMatch284/1 -> mul_Dot Product9_dotp_15/1(In1)
  t23/6 -> mul_Dot Product8_dotp_5/2(In2)
  t29/9 -> mul_Dot Product11_dotp_8/2(In2)
  Tapped Delay/1 -> Delay_Switch/1
  Dot Product1311/1(Out1) -> Dot Product1312/2(In2)
  mul_Dot Product2_dotp_8/1(Out1) -> delayMatch96/1
  delayMatch396/1 -> Dot Product128/1(In1)
  Dot Product910/1(Out1) -> Dot Product911/2(In2)
  Dot Product311/1(Out1) -> Dot Product312/2(In2)
  delayMatch229/1 -> mul_Dot Product7_dotp_10/1(In1)
  mul_Dot Product2_dotp_2/1(Out1) -> delayMatch90/1
  t15/14 -> mul_Dot Product4_dotp_13/2(In2)
  t35/12 -> mul_Dot Product14_dotp_11/2(In2)
  t24/16 -> delayMatch284/1
  Dot Product36/1(Out1) -> Dot Product37/2(In2)
  mul_Dot Product8_dotp_14/1(Out1) -> delayMatch282/1
  delayMatch75/1 -> mul_Dot Product2_dotp_14/1(In1)
  Dot Product1110/1(Out1) -> Dot Product1111/2(In2)
  delayMatch436/1 -> mul_Dot Product14_dotp_13/1(In1)
  t37/8 -> mul_Dot Product15_dotp_7/2(In2)
  mul_Dot Product4_dotp_0/1(Out1) -> Dot Product41/2(In2)
  delayMatch420/1 -> Dot Product132/1(In1)
  Unit Delay Enabled Synchronous22_lowered/1 -> Delay_Switch/3, in0_repeat/1
  t9/6 -> mul_Dot Product1_dotp_5/2(In2)
  t23/7 -> mul_Dot Product8_dotp_6/2(In2)
  t29/8 -> mul_Dot Product11_dotp_7/2(In2)
  t15/9 -> mul_Dot Product4_dotp_8/2(In2)
  t22/1 -> delayMatch269/1
  t29/16 -> mul_Dot Product11_dotp_15/2(In2)
  t29/10 -> mul_Dot Product11_dotp_9/2(In2)
  t8/2 -> delayMatch58/1
  t22/3 -> delayMatch267/1
  t7/15 -> mul_Dot Product_dotp_14/2(In2)
  t12/16 -> delayMatch104/1
  t29/13 -> mul_Dot Product11_dotp_12/2(In2)
  t22/4 -> delayMatch266/1
  mul_Dot Product7_dotp_0/1(Out1) -> Dot Product71/2(In2)
  mul_Dot Product10_dotp_10/1(Out1) -> delayMatch338/1
  D/1 -> in3_repeat1/1
  t8/1 -> delayMatch59/1
  Selector11/1 -> t28/1
  mul_Dot Product12_dotp_14/1(Out1) -> delayMatch402/1
  t15/16 -> mul_Dot Product4_dotp_15/2(In2)
  mul_Dot Product1_dotp_0/1(Out1) -> Dot Product15/2(In2)
  Dot Product515/1(Out1) -> mux1/6
  delayMatch352/1 -> mul_Dot Product11_dotp_7/1(In1)
  t22/6 -> delayMatch264/1
  Dot Product32/1(Out1) -> Dot Product33/2(In2)
  mul_Dot Product14_dotp_9/1(Out1) -> delayMatch457/1
  t7/1 -> mul_Dot Product_dotp_0/2(In2)
  t22/12 -> delayMatch258/1
  t22/13 -> delayMatch257/1
  Dot Product58/1(Out1) -> Dot Product59/2(In2)
  Dot Product1512/1(Out1) -> Dot Product1513/2(In2)
  t27/3 -> mul_Dot Product10_dotp_2/2(In2)
  t8/10 -> delayMatch50/1
  mul_Dot Product6_dotp_0/1(Out1) -> Dot Product61/2(In2)
  delayMatch113/1 -> mul_Dot Product3_dotp_6/1(In1)
  delayMatch198/1 -> mul_Dot Product6_dotp_11/1(In1)
  t10/7 -> delayMatch83/1
  delayMatch5/1 -> mux2/8
  Dot Product123/1(Out1) -> Dot Product124/2(In2)
  Dot Product74/1(Out1) -> Dot Product75/2(In2)
  delayMatch333/1 -> Dot Product105/1(In1)
  t20/1 -> delayMatch239/1
  Dot Product141/1(Out1) -> Dot Product142/2(In2)
  Dot Product513/1(Out1) -> Dot Product514/2(In2)
  Dot Product1114/1(Out1) -> Dot Product1115/2(In2)
  delayMatch171/1 -> mul_Dot Product5_dotp_8/1(In1)
  Dot Product1212/1(Out1) -> Dot Product1213/2(In2)
  t13/4 -> mul_Dot Product3_dotp_3/2(In2)
  t35/2 -> mul_Dot Product14_dotp_1/2(In2)
  delayMatch421/1 -> Dot Product133/1(In1)
  t3/7 -> Mux4_out1_6_term6/1
  t20/3 -> delayMatch237/1
  t20/4 -> delayMatch236/1
  delayMatch476/1 -> mul_Dot Product15_dotp_3/1(In1)
  t20/5 -> delayMatch235/1
  t18/2 -> delayMatch208/1
  t20/7 -> delayMatch233/1
  Dot Product158/1(Out1) -> Dot Product159/2(In2)
  delayMatch26/1 -> mul_Dot Product_dotp_3/1(In1)
  Dot Product113/1(Out1) -> Dot Product114/2(In2)
  t19/15 -> mul_Dot Product6_dotp_14/2(In2)
  Dot Product313/1(Out1) -> Dot Product314/2(In2)
  t15/2 -> mul_Dot Product4_dotp_1/2(In2)
  Dot Product312/1(Out1) -> Dot Product313/2(In2)
  Dot Product24/1(Out1) -> Dot Product25/2(In2)
  Dot Product1515/1(Out1) -> mux1/16
  t20/11 -> delayMatch229/1
  delayMatch221/1 -> Dot Product613/1(In1)
  delayMatch27/1 -> mul_Dot Product_dotp_2/1(In1)
  mul_Dot Product_dotp_3/1(Out1) -> delayMatch31/1
  t6/9 -> delayMatch21/1
  t19/3 -> mul_Dot Product6_dotp_2/2(In2)
  Dot Product1210/1(Out1) -> Dot Product1211/2(In2)
  t17/12 -> mul_Dot Product5_dotp_11/2(In2)
  t20/15 -> delayMatch225/1
  delayMatch367/1 -> Dot Product1118/1(In1)
  delayMatch16/1 -> mul_Dot Product_dotp_13/1(In1)
  t21/9 -> mul_Dot Product7_dotp_8/2(In2)
  t37/2 -> mul_Dot Product15_dotp_1/2(In2)
  delayMatch169/1 -> mul_Dot Product5_dotp_10/1(In1)
  delayMatch254/1 -> mul_Dot Product8_dotp_15/1(In1)
  t20/16 -> delayMatch224/1
  Dot Product64/1(Out1) -> Dot Product65/2(In2)
  Dot Product75/1(Out1) -> Dot Product76/2(In2)
  delayMatch195/1 -> mul_Dot Product6_dotp_14/1(In1)
  delayMatch80/1 -> mul_Dot Product2_dotp_9/1(In1)
  delayMatch303/1 -> Dot Product95/1(In1)
  t14/7 -> delayMatch143/1
  t17/3 -> mul_Dot Product5_dotp_2/2(In2)
  t31/2 -> mul_Dot Product12_dotp_1/2(In2)
  delayMatch309/1 -> Dot Product911/1(In1)
  Dot Product4/1(Out1) -> Dot Product5/2(In2)
  delayMatch471/1 -> mul_Dot Product15_dotp_8/1(In1)
  Dot Product51/1(Out1) -> Dot Product52/2(In2)
  Dot Product108/1(Out1) -> Dot Product109/2(In2)
  delayMatch14/1 -> mul_Dot Product_dotp_15/1(In1)
  t33/7 -> mul_Dot Product13_dotp_6/2(In2)
  t18/6 -> delayMatch204/1
  delayMatch11/1 -> mux2/14
  t18/7 -> delayMatch203/1
  t6/11 -> delayMatch19/1
  delayMatch102/1 -> Dot Product214/1(In1)
  t25/6 -> mul_Dot Product9_dotp_5/2(In2)
  Dot Product911/1(Out1) -> Dot Product912/2(In2)
  t31/1 -> mul_Dot Product12_dotp_0/2(In2)
  delayMatch167/1 -> mul_Dot Product5_dotp_12/1(In1)
  Dot Product91/1(Out1) -> Dot Product92/2(In2)
  Dot Product26/1(Out1) -> Dot Product27/2(In2)
  mul_Dot Product13_dotp_13/1(Out1) -> delayMatch431/1
  mul_Dot Product5_dotp_13/1(Out1) -> delayMatch191/1
  delayMatch446/1 -> mul_Dot Product14_dotp_3/1(In1)
  delayMatch21/1 -> mul_Dot Product_dotp_8/1(In1)
  delayMatch259/1 -> mul_Dot Product8_dotp_10/1(In1)
  Dot Product11/1(Out1) -> Dot Product12/2(In2)
  t12/7 -> delayMatch113/1
  t16/5 -> delayMatch175/1
  t18/12 -> delayMatch198/1
  t12/6 -> delayMatch114/1
  t18/13 -> delayMatch197/1
  t11/7 -> mul_Dot Product2_dotp_6/2(In2)
  t33/5 -> mul_Dot Product13_dotp_4/2(In2)
  delayMatch397/1 -> Dot Product129/1(In1)
  delayMatch493/1 -> Dot Product1515/1(In1)
  delayMatch457/1 -> Dot Product149/1(In1)
  delayMatch260/1 -> mul_Dot Product8_dotp_9/1(In1)
  t18/15 -> delayMatch195/1
  t8/11 -> delayMatch49/1
  t16/4 -> delayMatch176/1
  delayMatch401/1 -> Dot Product1213/1(In1)
  t16/10 -> delayMatch170/1
  mul_Dot Product11_dotp_14/1(Out1) -> delayMatch372/1
  Dot Product87/1(Out1) -> Dot Product88/2(In2)
  delayMatch203/1 -> mul_Dot Product6_dotp_6/1(In1)
  mul_Dot Product1_dotp_11/1(Out1) -> delayMatch69/1
  Dot Product111/1(Out1) -> Dot Product112/2(In2)
  t16/11 -> delayMatch169/1
  mul_Dot Product6_dotp_14/1(Out1) -> delayMatch222/1
  t10/1 -> delayMatch89/1
  t14/4 -> delayMatch146/1
  delayMatch127/1 -> Dot Product39/1(In1)
  t14/5 -> delayMatch145/1
  t21/1 -> mul_Dot Product7_dotp_0/2(In2)
  t14/8 -> delayMatch142/1
  delayMatch393/1 -> Dot Product125/1(In1)
  delayMatch374/1 -> mul_Dot Product12_dotp_15/1(In1)
  mul_Dot Product12_dotp_3/1(Out1) -> delayMatch391/1
  t9/13 -> mul_Dot Product1_dotp_12/2(In2)
  t14/10 -> delayMatch140/1
  t17/10 -> mul_Dot Product5_dotp_9/2(In2)
  delayMatch139/1 -> mul_Dot Product4_dotp_10/1(In1)
  Dot Product144/1(Out1) -> Dot Product145/2(In2)
  t9/12 -> mul_Dot Product1_dotp_11/2(In2)
  t14/11 -> delayMatch139/1
  t17/11 -> mul_Dot Product5_dotp_10/2(In2)
  t31/10 -> mul_Dot Product12_dotp_9/2(In2)
  t25/4 -> mul_Dot Product9_dotp_3/2(In2)
  Selector6/1 -> t18/1
  t17/9 -> mul_Dot Product5_dotp_8/2(In2)
  t10/16 -> delayMatch74/1
  Selector5/1 -> t16/1
  Dot Product9/1(Out1) -> Dot Product10/2(In2)
  delayMatch217/1 -> Dot Product69/1(In1)
  delayMatch305/1 -> Dot Product97/1(In1)
  t14/16 -> delayMatch134/1
  Dot Product73/1(Out1) -> Dot Product74/2(In2)
  t12/1 -> delayMatch119/1
  mul_Dot Product3_dotp_13/1(Out1) -> delayMatch131/1
  mul_Dot Product_dotp_14/1(Out1) -> delayMatch42/1
  delayMatch298/1 -> mul_Dot Product9_dotp_1/1(In1)
  in0_repeat/1 -> Selector15/1, Selector12/1, Selector11/1, Selector7/1, Selector5/1, Selector4/1, Selector/1, Selector6/1, Selector1/1, Selector2/1, Selector14/1, Selector8/1, Selector9/1, Selector13/1, Selector10/1, Selector3/1
  t4/3 -> mux2/3
  delayMatch466/1 -> mul_Dot Product15_dotp_13/1(In1)
  Dot Product28/1(Out1) -> Dot Product29/2(In2)
  Dot Product1213/1(Out1) -> Dot Product1214/2(In2)
  t19/5 -> mul_Dot Product6_dotp_4/2(In2)
  t12/12 -> delayMatch108/1
  t23/9 -> mul_Dot Product8_dotp_8/2(In2)
  t29/2 -> mul_Dot Product11_dotp_1/2(In2)
  t10/2 -> delayMatch88/1
  delayMatch404/1 -> mul_Dot Product13_dotp_15/1(In1)
  t11/12 -> mul_Dot Product2_dotp_11/2(In2)
  t33/2 -> mul_Dot Product13_dotp_1/2(In2)
  t15/12 -> mul_Dot Product4_dotp_11/2(In2)
  t13/13 -> mul_Dot Product3_dotp_12/2(In2)
  t21/14 -> mul_Dot Product7_dotp_13/2(In2)
  Dot Product614/1(Out1) -> Dot Product615/2(In2)
  t27/12 -> mul_Dot Product10_dotp_11/2(In2)
  delayMatch135/1 -> mul_Dot Product4_dotp_14/1(In1)
  t13/15 -> mul_Dot Product3_dotp_14/2(In2)
  t10/8 -> delayMatch82/1
  in4_repeat/1 -> delayMatch495/1
  delayMatch165/1 -> mul_Dot Product5_dotp_14/1(In1)
  delayMatch99/1 -> Dot Product211/1(In1)
  delayMatch345/1 -> mul_Dot Product11_dotp_14/1(In1)
  t10/14 -> delayMatch76/1
  t35/7 -> mul_Dot Product14_dotp_6/2(In2)
  t10/15 -> delayMatch75/1
  delayMatch431/1 -> Dot Product1313/1(In1)
  delayMatch190/1 -> Dot Product512/1(In1)
  delayMatch105/1 -> mul_Dot Product3_dotp_14/1(In1)
  delayMatch387/1 -> mul_Dot Product12_dotp_2/1(In1)
  t8/16 -> delayMatch44/1
  t6/1 -> delayMatch29/1
  delayMatch313/1 -> Dot Product915/1(In1)
  t6/10 -> delayMatch20/1
  delayMatch205/1 -> mul_Dot Product6_dotp_4/1(In1)
  delayMatch224/1 -> mul_Dot Product7_dotp_15/1(In1)
  delayMatch211/1 -> Dot Product63/1(In1)
  mul_Dot Product9_dotp_0/1(Out1) -> Dot Product91/2(In2)
  t5/7 -> delayMatch9/1
  Dot Product85/1(Out1) -> Dot Product86/2(In2)
  t6/12 -> delayMatch18/1
  Dot Product145/1(Out1) -> Dot Product146/2(In2)
  delayMatch413/1 -> mul_Dot Product13_dotp_6/1(In1)
  t6/13 -> delayMatch17/1
  Dot Product155/1(Out1) -> Dot Product156/2(In2)
  mul_Dot Product7_dotp_6/1(Out1) -> delayMatch244/1
  delayMatch290/1 -> mul_Dot Product9_dotp_9/1(In1)
  delayMatch252/1 -> Dot Product714/1(In1)
  delayMatch449/1 -> mul_Dot Product14_dotp_0/1(In1)
  t6/14 -> delayMatch16/1
  Dot Product56/1(Out1) -> Dot Product57/2(In2)
  delayMatch149/1 -> mul_Dot Product4_dotp_0/1(In1)
  mul_Dot Product12_dotp_11/1(Out1) -> delayMatch399/1
  t11/13 -> mul_Dot Product2_dotp_12/2(In2)
  t6/16 -> delayMatch14/1
  t5/9 -> delayMatch11/1
  mul_Dot Product15_dotp_13/1(Out1) -> delayMatch491/1
  t9/7 -> mul_Dot Product1_dotp_6/2(In2)
  t11/6 -> mul_Dot Product2_dotp_5/2(In2)
  delayMatch369/1 -> Dot Product1120/1(In1)
  mul_Dot Product5_dotp_4/1(Out1) -> delayMatch182/1
  mul_Dot Product9_dotp_12/1(Out1) -> delayMatch310/1
  delayMatch495/1 -> t39/2, t39/1
  mul_Dot Product13_dotp_9/1(Out1) -> delayMatch427/1
  t31/16 -> mul_Dot Product12_dotp_15/2(In2)
  delayMatch450/1 -> Dot Product142/1(In1)
  delayMatch51/1 -> mul_Dot Product1_dotp_8/1(In1)
  t5/5 -> delayMatch7/1
  t5/4 -> delayMatch6/1
  Dot Product77/1(Out1) -> Dot Product78/2(In2)
  mi/1 -> PWM Generator/1(mod_index)
  t5/2 -> delayMatch4/1
  t5/1 -> delayMatch3/1
  mul_Dot Product15_dotp_15/1(Out1) -> delayMatch493/1
  t27/10 -> mul_Dot Product10_dotp_9/2(In2)
  t21/12 -> mul_Dot Product7_dotp_11/2(In2)
  Dot Product151/1(Out1) -> Dot Product152/2(In2)
  delayMatch383/1 -> mul_Dot Product12_dotp_6/1(In1)
  Dot Product57/1(Out1) -> Dot Product58/2(In2)
  delayMatch153/1 -> Dot Product45/1(In1)
  delayMatch238/1 -> mul_Dot Product7_dotp_1/1(In1)
  mul_Dot Product15_dotp_12/1(Out1) -> delayMatch490/1
  Dot Product53/1(Out1) -> Dot Product54/2(In2)
  delayMatch343/1 -> Dot Product1015/1(In1)
  Dot Product1314/1(Out1) -> Dot Product1315/2(In2)
  delayMatch439/1 -> mul_Dot Product14_dotp_10/1(In1)
  Dot Product1510/1(Out1) -> Dot Product1511/2(In2)
  mul_Dot Product15_dotp_9/1(Out1) -> delayMatch487/1
  t23/16 -> mul_Dot Product8_dotp_15/2(In2)
  t31/7 -> mul_Dot Product12_dotp_6/2(In2)
  t35/14 -> mul_Dot Product14_dotp_13/2(In2)
  t21/15 -> mul_Dot Product7_dotp_14/2(In2)
  Dot Product714/1(Out1) -> Dot Product715/2(In2)
  delayMatch24/1 -> mul_Dot Product_dotp_5/1(In1)
  Dot Product210/1(Out1) -> Dot Product211/2(In2)
  mul_Dot Product9_dotp_5/1(Out1) -> delayMatch303/1
  Dot Product157/1(Out1) -> Dot Product158/2(In2)
  t35/13 -> mul_Dot Product14_dotp_12/2(In2)
  mul_Dot Product6_dotp_2/1(Out1) -> delayMatch210/1
  t37/13 -> mul_Dot Product15_dotp_12/2(In2)
  mul_Dot Product6_dotp_10/1(Out1) -> delayMatch218/1
  Dot Product124/1(Out1) -> Dot Product125/2(In2)
  mul_Dot Product11_dotp_13/1(Out1) -> delayMatch371/1
  mul_Dot Product14_dotp_12/1(Out1) -> delayMatch460/1
  delayMatch419/1 -> mul_Dot Product13_dotp_0/1(In1)
  delayMatch451/1 -> Dot Product143/1(In1)
  Dot Product152/1(Out1) -> Dot Product153/2(In2)
  t25/9 -> mul_Dot Product9_dotp_8/2(In2)
  mul_Dot Product15_dotp_2/1(Out1) -> delayMatch480/1
  Dot Product7/1(Out1) -> Dot Product8/2(In2)
  mul_Dot Product15_dotp_1/1(Out1) -> Dot Product151/1(In1)
  t27/13 -> mul_Dot Product10_dotp_12/2(In2)
  Dot Product1214/1(Out1) -> Dot Product1215/2(In2)
  Dot Product1116/1(Out1) -> Dot Product1117/2(In2)
  Dot Product713/1(Out1) -> Dot Product714/2(In2)
  t37/14 -> mul_Dot Product15_dotp_13/2(In2)
  delayMatch151/1 -> Dot Product43/1(In1)
  Dot Product62/1(Out1) -> Dot Product63/2(In2)
  delayMatch412/1 -> mul_Dot Product13_dotp_7/1(In1)
  delayMatch213/1 -> Dot Product65/1(In1)
  mul_Dot Product9_dotp_3/1(Out1) -> delayMatch301/1
  delayMatch409/1 -> mul_Dot Product13_dotp_10/1(In1)
  t27/16 -> mul_Dot Product10_dotp_15/2(In2)
  delayMatch379/1 -> mul_Dot Product12_dotp_10/1(In1)
  Dot Product143/1(Out1) -> Dot Product144/2(In2)
  t37/3 -> mul_Dot Product15_dotp_2/2(In2)
  Dot Product23/1(Out1) -> Dot Product24/2(In2)
  delayMatch306/1 -> Dot Product98/1(In1)
  t15/3 -> mul_Dot Product4_dotp_2/2(In2)
  t19/14 -> mul_Dot Product6_dotp_13/2(In2)
  delayMatch236/1 -> mul_Dot Product7_dotp_3/1(In1)
  mul_Dot Product11_dotp_1/1(Out1) -> Dot Product1110/1(In1)
  delayMatch465/1 -> mul_Dot Product15_dotp_14/1(In1)
  Dot Product142/1(Out1) -> Dot Product143/2(In2)
  delayMatch311/1 -> Dot Product913/1(In1)
  Goto/1 -> From/1
  t21/10 -> mul_Dot Product7_dotp_9/2(In2)
  t27/15 -> mul_Dot Product10_dotp_14/2(In2)
  mul_Dot Product14_dotp_1/1(Out1) -> Dot Product141/1(In1)
  Dot Product/1(Out1) -> Dot Product1/2(In2)
  delayMatch63/1 -> Dot Product19/1(In1)
  in3_repeat/1 -> Index Vector_dtc_comp/1
  delayMatch131/1 -> Dot Product313/1(In1)
  Dot Product1315/1(Out1) -> mux1/14
  t4/4 -> mux2/4
  Selector10/1 -> t26/1
  delayMatch380/1 -> mul_Dot Product12_dotp_9/1(In1)
  Dot Product1313/1(Out1) -> Dot Product1314/2(In2)
  delayMatch475/1 -> mul_Dot Product15_dotp_4/1(In1)
  Dot Product1312/1(Out1) -> Dot Product1313/2(In2)
  delayMatch398/1 -> Dot Product1210/1(In1)
  Dot Product1123/1(Out1) -> Dot Product1124/2(In2)
  delayMatch136/1 -> mul_Dot Product4_dotp_13/1(In1)
  t7/5 -> mul_Dot Product_dotp_4/2(In2)
  delayMatch174/1 -> mul_Dot Product5_dotp_5/1(In1)
  Dot Product138/1(Out1) -> Dot Product139/2(In2)
  mul_Dot Product5_dotp_0/1(Out1) -> Dot Product51/2(In2)
  Dot Product84/1(Out1) -> Dot Product85/2(In2)
  Dot Product137/1(Out1) -> Dot Product138/2(In2)
  delayMatch19/1 -> mul_Dot Product_dotp_10/1(In1)
  t9/16 -> mul_Dot Product1_dotp_15/2(In2)
  t31/6 -> mul_Dot Product12_dotp_5/2(In2)
  mul_Dot Product13_dotp_15/1(Out1) -> delayMatch433/1
  delayMatch323/1 -> mul_Dot Product10_dotp_6/1(In1)
  delayMatch285/1 -> mul_Dot Product9_dotp_14/1(In1)
  Dot Product25/1(Out1) -> Dot Product26/2(In2)
  Dot Product133/1(Out1) -> Dot Product134/2(In2)
  Dot Product131/1(Out1) -> Dot Product132/2(In2)
  t3/14 -> Mux4_out1_13_term13/1
  t11/15 -> mul_Dot Product2_dotp_14/2(In2)
  t33/13 -> mul_Dot Product13_dotp_12/2(In2)
  mul_Dot Product13_dotp_0/1(Out1) -> Dot Product131/2(In2)
  Dot Product98/1(Out1) -> Dot Product99/2(In2)
  Dot Product97/1(Out1) -> Dot Product98/2(In2)
  t37/15 -> mul_Dot Product15_dotp_14/2(In2)
  t23/5 -> mul_Dot Product8_dotp_4/2(In2)
  t33/15 -> mul_Dot Product13_dotp_14/2(In2)
  Dot Product1211/1(Out1) -> Dot Product1212/2(In2)
  delayMatch314/1 -> mul_Dot Product10_dotp_15/1(In1)
  delayMatch327/1 -> mul_Dot Product10_dotp_2/1(In1)
  Dot Product129/1(Out1) -> Dot Product1210/2(In2)
  Dot Product126/1(Out1) -> Dot Product127/2(In2)
  Dot Product1117/1(Out1) -> Dot Product1118/2(In2)
  Dot Product122/1(Out1) -> Dot Product123/2(In2)
  delayMatch249/1 -> Dot Product711/1(In1)
  mul_Dot Product12_dotp_1/1(Out1) -> Dot Product121/1(In1)
  Dot Product813/1(Out1) -> Dot Product814/2(In2)
  crp_out_delay/1 -> Delay/1
  Dot Product314/1(Out1) -> Dot Product315/2(In2)
  mul_Dot Product_dotp_7/1(Out1) -> delayMatch35/1
  delayMatch53/1 -> mul_Dot Product1_dotp_6/1(In1)
  delayMatch163/1 -> Dot Product415/1(In1)
  delayMatch294/1 -> mul_Dot Product9_dotp_5/1(In1)
  Dot Product1121/1(Out1) -> Dot Product1122/2(In2)
  Dot Product710/1(Out1) -> Dot Product711/2(In2)
  Dot Product1115/1(Out1) -> Dot Product1116/2(In2)
  delayMatch216/1 -> Dot Product68/1(In1)
  t23/13 -> mul_Dot Product8_dotp_12/2(In2)
  delayMatch318/1 -> mul_Dot Product10_dotp_11/1(In1)
  Dot Product14/1(Out1) -> mux1/1
  Dot Product1010/1(Out1) -> Dot Product1011/2(In2)
  t1/1 -> user_out_8sig/1
  mul_Dot Product11_dotp_0/1(Out1) -> Dot Product1110/2(In2)
  mul_Dot Product4_dotp_3/1(Out1) -> delayMatch151/1
  Dcnt/1 -> Compare To Constant/1(u)
  delayMatch178/1 -> mul_Dot Product5_dotp_1/1(In1)
  delayMatch389/1 -> mul_Dot Product12_dotp_0/1(In1)
  Dot Product1015/1(Out1) -> mux1/11
  delayMatch282/1 -> Dot Product814/1(In1)
  delayMatch441/1 -> mul_Dot Product14_dotp_8/1(In1)
  Selector15/1 -> t36/1
  delayMatch52/1 -> mul_Dot Product1_dotp_7/1(In1)
  delayMatch373/1 -> Dot Product1124/1(In1)
  Dot Product88/1(Out1) -> Dot Product89/2(In2)
  t13/10 -> mul_Dot Product3_dotp_9/2(In2)
  Dot Product1013/1(Out1) -> Dot Product1014/2(In2)
  delayMatch325/1 -> mul_Dot Product10_dotp_4/1(In1)
  Dot Product1011/1(Out1) -> Dot Product1012/2(In2)
  Dot Product96/1(Out1) -> Dot Product97/2(In2)
  t31/15 -> mul_Dot Product12_dotp_14/2(In2)
  delayMatch243/1 -> Dot Product75/1(In1)
  mul_Dot Product6_dotp_6/1(Out1) -> delayMatch214/1
  Dot Product107/1(Out1) -> Dot Product108/2(In2)
  Dot Product104/1(Out1) -> Dot Product105/2(In2)
  mul_Dot Product10_dotp_4/1(Out1) -> delayMatch332/1
  t25/11 -> mul_Dot Product9_dotp_10/2(In2)
  t11/10 -> mul_Dot Product2_dotp_9/2(In2)
  t33/8 -> mul_Dot Product13_dotp_7/2(In2)
  Dot Product101/1(Out1) -> Dot Product102/2(In2)
  delayMatch36/1 -> Dot Product7/1(In1)
  mul_Dot Product10_dotp_1/1(Out1) -> Dot Product101/1(In1)
  delayMatch155/1 -> Dot Product47/1(In1)
  mul_Dot Product3_dotp_1/1(Out1) -> Dot Product31/1(In1)
  Dot Product914/1(Out1) -> Dot Product915/2(In2)
  t23/14 -> mul_Dot Product8_dotp_13/2(In2)
  t31/13 -> mul_Dot Product12_dotp_12/2(In2)
  mul_Dot Product9_dotp_14/1(Out1) -> delayMatch312/1
  delayMatch41/1 -> Dot Product12/1(In1)
  delayMatch385/1 -> mul_Dot Product12_dotp_4/1(In1)
  Dot Product2/1(Out1) -> Dot Product3/2(In2)
  Dot Product1/1(Out1) -> Dot Product2/2(In2)
  Dot Product94/1(Out1) -> Dot Product95/2(In2)
  mul_Dot Product9_dotp_4/1(Out1) -> delayMatch302/1
  delayMatch443/1 -> mul_Dot Product14_dotp_6/1(In1)
  Dot Product815/1(Out1) -> mux1/9
  Dot Product814/1(Out1) -> Dot Product815/2(In2)
  delayMatch338/1 -> Dot Product1010/1(In1)
  mul_Dot Product8_dotp_12/1(Out1) -> delayMatch280/1
  delayMatch204/1 -> mul_Dot Product6_dotp_5/1(In1)
  Dot Product811/1(Out1) -> Dot Product812/2(In2)
  delayMatch360/1 -> Dot Product1111/1(In1)
  Dot Product810/1(Out1) -> Dot Product811/2(In2)
  mul_Dot Product7_dotp_15/1(Out1) -> delayMatch253/1
  delayMatch50/1 -> mul_Dot Product1_dotp_9/1(In1)
  t33/11 -> mul_Dot Product13_dotp_10/2(In2)
  Dot Product89/1(Out1) -> Dot Product810/2(In2)
  in2_repeat/1 -> t5/1
  delayMatch173/1 -> mul_Dot Product5_dotp_6/1(In1)
  mul_Dot Product8_dotp_9/1(Out1) -> delayMatch277/1
  t9/4 -> mul_Dot Product1_dotp_3/2(In2)
  t25/16 -> mul_Dot Product9_dotp_15/2(In2)
  t29/6 -> mul_Dot Product11_dotp_5/2(In2)
  Dot Product315/1(Out1) -> mux1/4
  delayMatch214/1 -> Dot Product66/1(In1)
  delayMatch129/1 -> Dot Product311/1(In1)
  delayMatch162/1 -> Dot Product414/1(In1)
  t37/10 -> mul_Dot Product15_dotp_9/2(In2)
  Dot Product81/1(Out1) -> Dot Product82/2(In2)
  delayMatch407/1 -> mul_Dot Product13_dotp_12/1(In1)
  delayMatch64/1 -> Dot Product110/1(In1)
  t15/8 -> mul_Dot Product4_dotp_7/2(In2)
  Dot Product16/1(Out1) -> Dot Product17/2(In2)
  Dot Product715/1(Out1) -> mux1/8
  Dot Product712/1(Out1) -> Dot Product713/2(In2)
  delayMatch69/1 -> Dot Product115/1(In1)
  delayMatch269/1 -> mul_Dot Product8_dotp_0/1(In1)
  t7/11 -> mul_Dot Product_dotp_10/2(In2)
  CrossICidx/1 -> LC vectorized/4(Xin_idx)
  Dot Product76/1(Out1) -> Dot Product77/2(In2)
  delayMatch66/1 -> Dot Product112/1(In1)
  t3/3 -> Demux_mux_1/3
  t23/8 -> mul_Dot Product8_dotp_7/2(In2)
  t29/3 -> mul_Dot Product11_dotp_2/2(In2)
  t25/13 -> mul_Dot Product9_dotp_12/2(In2)
  mul_Dot Product7_dotp_4/1(Out1) -> delayMatch242/1
  delayMatch356/1 -> mul_Dot Product11_dotp_3/1(In1)
  mul_Dot Product6_dotp_9/1(Out1) -> delayMatch217/1
  t29/7 -> mul_Dot Product11_dotp_6/2(In2)
  mul_Dot Product7_dotp_1/1(Out1) -> Dot Product71/1(In1)
  delayMatch324/1 -> mul_Dot Product10_dotp_5/1(In1)
  Dot Product615/1(Out1) -> mux1/7
  delayMatch152/1 -> Dot Product44/1(In1)
  delayMatch382/1 -> mul_Dot Product12_dotp_7/1(In1)
  delayMatch164/1 -> mul_Dot Product5_dotp_15/1(In1)
  Dot Product610/1(Out1) -> Dot Product611/2(In2)
  Dot Product512/1(Out1) -> Dot Product513/2(In2)
  Dot Product69/1(Out1) -> Dot Product610/2(In2)
  delayMatch492/1 -> Dot Product1514/1(In1)
  Dot Product68/1(Out1) -> Dot Product69/2(In2)
  t25/3 -> mul_Dot Product9_dotp_2/2(In2)
  t27/2 -> mul_Dot Product10_dotp_1/2(In2)
  t31/4 -> mul_Dot Product12_dotp_3/2(In2)
  Dot Product43/1(Out1) -> Dot Product44/2(In2)
  Dot Product511/1(Out1) -> Dot Product512/2(In2)
  delayMatch103/1 -> Dot Product215/1(In1)
  Dot Product65/1(Out1) -> Dot Product66/2(In2)
  Dot Product63/1(Out1) -> Dot Product64/2(In2)
  delayMatch344/1 -> mul_Dot Product11_dotp_15/1(In1)
  t13/16 -> mul_Dot Product3_dotp_15/2(In2)
  t35/6 -> mul_Dot Product14_dotp_5/2(In2)
  mul_Dot Product11_dotp_8/1(Out1) -> delayMatch366/1
  delayMatch410/1 -> mul_Dot Product13_dotp_9/1(In1)
  delayMatch89/1 -> mul_Dot Product2_dotp_0/1(In1)
  t11/4 -> mul_Dot Product2_dotp_3/2(In2)
  t23/10 -> mul_Dot Product8_dotp_9/2(In2)
  t29/5 -> mul_Dot Product11_dotp_4/2(In2)
  t9/3 -> mul_Dot Product1_dotp_2/2(In2)
  mul_Dot Product4_dotp_13/1(Out1) -> delayMatch161/1
  mul_Dot Product5_dotp_12/1(Out1) -> delayMatch190/1
  delayMatch364/1 -> Dot Product1115/1(In1)
  delayMatch293/1 -> mul_Dot Product9_dotp_6/1(In1)
  Dot Product59/1(Out1) -> Dot Product510/2(In2)
  mul_Dot Product5_dotp_9/1(Out1) -> delayMatch187/1
  t17/15 -> mul_Dot Product5_dotp_14/2(In2)
  delayMatch279/1 -> Dot Product811/1(In1)
  Dot Product19/1(Out1) -> Dot Product110/2(In2)
  delayMatch395/1 -> Dot Product127/1(In1)
  t7/9 -> mul_Dot Product_dotp_8/2(In2)
  Dot Product52/1(Out1) -> Dot Product53/2(In2)
  Dot Product413/1(Out1) -> Dot Product414/2(In2)
  delayMatch422/1 -> Dot Product134/1(In1)
  Dot Product44/1(Out1) -> Dot Product45/2(In2)
  delayMatch464/1 -> mul_Dot Product15_dotp_15/1(In1)
  delayMatch237/1 -> mul_Dot Product7_dotp_2/1(In1)
  delayMatch353/1 -> mul_Dot Product11_dotp_6/1(In1)
  delayMatch72/1 -> Dot Product118/1(In1)
  Dot Product49/1(Out1) -> Dot Product410/2(In2)
  Dot Product37/1(Out1) -> Dot Product38/2(In2)
  Dot Product47/1(Out1) -> Dot Product48/2(In2)
  mul_Dot Product1_dotp_7/1(Out1) -> delayMatch65/1
  Dot Product45/1(Out1) -> Dot Product46/2(In2)
  delayMatch141/1 -> mul_Dot Product4_dotp_8/1(In1)
  delayMatch122/1 -> Dot Product34/1(In1)
  mul_Dot Product4_dotp_1/1(Out1) -> Dot Product41/1(In1)
  mul_Dot Product2_dotp_15/1(Out1) -> delayMatch103/1
  delayMatch347/1 -> mul_Dot Product11_dotp_12/1(In1)
  Dot Product310/1(Out1) -> Dot Product311/2(In2)
  mul_Dot Product3_dotp_8/1(Out1) -> delayMatch126/1
  Dot Product35/1(Out1) -> Dot Product36/2(In2)
  Dot Product34/1(Out1) -> Dot Product35/2(In2)
  delayMatch115/1 -> mul_Dot Product3_dotp_4/1(In1)
  mul_Dot Product6_dotp_12/1(Out1) -> delayMatch220/1
  mul_Dot Product3_dotp_2/1(Out1) -> delayMatch120/1
  t7/10 -> mul_Dot Product_dotp_9/2(In2)
  Dot Product214/1(Out1) -> Dot Product215/2(In2)
  delayMatch403/1 -> Dot Product1215/1(In1)
  delayMatch65/1 -> Dot Product111/1(In1)
  Selector12/1 -> t30/1
  t23/11 -> mul_Dot Product8_dotp_10/2(In2)
  t29/4 -> mul_Dot Product11_dotp_3/2(In2)
  Dot Product213/1(Out1) -> Dot Product214/2(In2)
  delayMatch112/1 -> mul_Dot Product3_dotp_7/1(In1)
  Dot Product27/1(Out1) -> Dot Product28/2(In2)
  t35/16 -> mul_Dot Product14_dotp_15/2(In2)
  delayMatch88/1 -> mul_Dot Product2_dotp_1/1(In1)
  Dot Product21/1(Out1) -> Dot Product22/2(In2)
  Dot Product119/1(Out1) -> mux1/2
  t7/13 -> mul_Dot Product_dotp_12/2(In2)
  delayMatch71/1 -> Dot Product117/1(In1)
  Dot Product118/1(Out1) -> Dot Product119/2(In2)
  Dot Product13/1(Out1) -> Dot Product14/2(In2)
  delayMatch184/1 -> Dot Product56/1(In1)
  delayMatch350/1 -> mul_Dot Product11_dotp_9/1(In1)
  Dot Product117/1(Out1) -> Dot Product118/2(In2)
  Dot Product114/1(Out1) -> Dot Product115/2(In2)
  mul_Dot Product1_dotp_4/1(Out1) -> delayMatch62/1
  mul_Dot Product1_dotp_1/1(Out1) -> Dot Product15/1(In1)
  delayMatch251/1 -> Dot Product713/1(In1)
  mul_Dot Product_dotp_15/1(Out1) -> delayMatch43/1
  t27/6 -> mul_Dot Product10_dotp_5/2(In2)
  t21/16 -> mul_Dot Product7_dotp_15/2(In2)
  Dot Product8/1(Out1) -> Dot Product9/2(In2)
  delayMatch148/1 -> mul_Dot Product4_dotp_1/1(In1)
  Dot Product3/1(Out1) -> Dot Product4/2(In2)
  mul_Dot Product13_dotp_6/1(Out1) -> delayMatch424/1
  t37/9 -> mul_Dot Product15_dotp_8/2(In2)
  t33/16 -> mul_Dot Product13_dotp_15/2(In2)
  delayMatch201/1 -> mul_Dot Product6_dotp_8/1(In1)
  mul_Dot Product_dotp_1/1(Out1) -> Dot Product/1(In1)
  delayMatch482/1 -> Dot Product154/1(In1)
  delayMatch79/1 -> mul_Dot Product2_dotp_10/1(In1)
  mul_Dot Product_dotp_0/1(Out1) -> Dot Product/2(In2)
  delayMatch491/1 -> Dot Product1513/1(In1)
  delayMatch485/1 -> Dot Product157/1(In1)
  delayMatch156/1 -> Dot Product48/1(In1)
  delayMatch42/1 -> Dot Product13/1(In1)
  delayMatch386/1 -> mul_Dot Product12_dotp_3/1(In1)
  delayMatch480/1 -> Dot Product152/1(In1)
  delayMatch440/1 -> mul_Dot Product14_dotp_9/1(In1)
  t21/5 -> mul_Dot Product7_dotp_4/2(In2)
  mul_Dot Product2_dotp_5/1(Out1) -> delayMatch93/1
  t37/16 -> mul_Dot Product15_dotp_15/2(In2)
  delayMatch73/1 -> Dot Product119/1(In1)
  t37/12 -> mul_Dot Product15_dotp_11/2(In2)
  t37/6 -> mul_Dot Product15_dotp_5/2(In2)
  mul_Dot Product11_dotp_5/1(Out1) -> delayMatch363/1
  delayMatch18/1 -> mul_Dot Product_dotp_11/1(In1)
  t37/4 -> mul_Dot Product15_dotp_3/2(In2)
  t13/1 -> mul_Dot Product3_dotp_0/2(In2)
  delayMatch467/1 -> mul_Dot Product15_dotp_12/1(In1)
  delayMatch470/1 -> mul_Dot Product15_dotp_9/1(In1)
  minus_g/1 -> LC vectorized/2(minus_g)
  delayMatch244/1 -> Dot Product76/1(In1)
  delayMatch473/1 -> mul_Dot Product15_dotp_6/1(In1)
  delayMatch218/1 -> Dot Product610/1(In1)
  t35/11 -> mul_Dot Product14_dotp_10/2(In2)
  PWMsteps/1 -> PWM Generator/2(steps)
  delayMatch433/1 -> Dot Product1315/1(In1)
  t35/10 -> mul_Dot Product14_dotp_9/2(In2)
  delayMatch126/1 -> Dot Product38/1(In1)
  t11/2 -> mul_Dot Product2_dotp_1/2(In2)
  t13/3 -> mul_Dot Product3_dotp_2/2(In2)
  t35/1 -> mul_Dot Product14_dotp_0/2(In2)
  delayMatch130/1 -> Dot Product312/1(In1)
  Selector7/1 -> t20/1
  delayMatch435/1 -> mul_Dot Product14_dotp_14/1(In1)
  delayMatch437/1 -> mul_Dot Product14_dotp_12/1(In1)
  delayMatch438/1 -> mul_Dot Product14_dotp_11/1(In1)
  delayMatch38/1 -> Dot Product9/1(In1)
  LC vectorized/1(Hist) -> Goto/1
  mul_Dot Product11_dotp_3/1(Out1) -> delayMatch361/1
  delayMatch445/1 -> mul_Dot Product14_dotp_4/1(In1)
  delayMatch448/1 -> mul_Dot Product14_dotp_1/1(In1)
  delayMatch432/1 -> Dot Product1314/1(In1)
  delayMatch428/1 -> Dot Product1310/1(In1)
  t7/3 -> mul_Dot Product_dotp_2/2(In2)
  t33/10 -> mul_Dot Product13_dotp_9/2(In2)
  delayMatch255/1 -> mul_Dot Product8_dotp_14/1(In1)
  t33/4 -> mul_Dot Product13_dotp_3/2(In2)
  delayMatch275/1 -> Dot Product87/1(In1)
  delayMatch408/1 -> mul_Dot Product13_dotp_11/1(In1)
  Delay_absorbed/1 -> Tapped Delay/1
  delayMatch417/1 -> mul_Dot Product13_dotp_2/1(In1)
  delayMatch496/1 -> user_out_clk/1
  delayMatch140/1 -> mul_Dot Product4_dotp_9/1(In1)
  delayMatch402/1 -> Dot Product1214/1(In1)
  mul_Dot Product10_dotp_13/1(Out1) -> delayMatch341/1
  delayMatch390/1 -> Dot Product122/1(In1)
  mul_Dot Product15_dotp_6/1(Out1) -> delayMatch484/1
  t31/14 -> mul_Dot Product12_dotp_13/2(In2)
  delayMatch316/1 -> mul_Dot Product10_dotp_13/1(In1)
  t31/8 -> mul_Dot Product12_dotp_7/2(In2)
  Selector4/1 -> t14/1
  t25/2 -> mul_Dot Product9_dotp_1/2(In2)
  t31/5 -> mul_Dot Product12_dotp_4/2(In2)
  t31/3 -> mul_Dot Product12_dotp_2/2(In2)
  delayMatch375/1 -> mul_Dot Product12_dotp_14/1(In1)
  delayMatch376/1 -> mul_Dot Product12_dotp_13/1(In1)
  delayMatch366/1 -> Dot Product1117/1(In1)
  delayMatch168/1 -> mul_Dot Product5_dotp_11/1(In1)
  delayMatch40/1 -> Dot Product11/1(In1)
  delayMatch384/1 -> mul_Dot Product12_dotp_5/1(In1)
  delayMatch372/1 -> Dot Product1123/1(In1)
  delayMatch371/1 -> Dot Product1122/1(In1)
  delayMatch363/1 -> Dot Product1114/1(In1)
  delayMatch361/1 -> Dot Product1112/1(In1)
  t29/15 -> mul_Dot Product11_dotp_14/2(In2)
  delayMatch346/1 -> mul_Dot Product11_dotp_13/1(In1)
  delayMatch147/1 -> mul_Dot Product4_dotp_2/1(In1)
  delayMatch351/1 -> mul_Dot Product11_dotp_8/1(In1)
  delayMatch359/1 -> mul_Dot Product11_dotp_0/1(In1)
  delayMatch200/1 -> mul_Dot Product6_dotp_9/1(In1)
  delayMatch334/1 -> Dot Product106/1(In1)
  t27/14 -> mul_Dot Product10_dotp_13/2(In2)
  t27/11 -> mul_Dot Product10_dotp_10/2(In2)
  t21/11 -> mul_Dot Product7_dotp_10/2(In2)
  t27/9 -> mul_Dot Product10_dotp_8/2(In2)
  t19/2 -> mul_Dot Product6_dotp_1/2(In2)
  delayMatch100/1 -> Dot Product212/1(In1)
  t27/8 -> mul_Dot Product10_dotp_7/2(In2)
  t13/14 -> mul_Dot Product3_dotp_13/2(In2)
  t27/7 -> mul_Dot Product10_dotp_6/2(In2)
  t27/5 -> mul_Dot Product10_dotp_4/2(In2)
  delayMatch134/1 -> mul_Dot Product4_dotp_15/1(In1)
  t21/6 -> mul_Dot Product7_dotp_5/2(In2)
  delayMatch240/1 -> Dot Product72/1(In1)
  t27/4 -> mul_Dot Product10_dotp_3/2(In2)
  delayMatch315/1 -> mul_Dot Product10_dotp_14/1(In1)
  delayMatch304/1 -> Dot Product96/1(In1)
  delayMatch317/1 -> mul_Dot Product10_dotp_12/1(In1)
  delayMatch183/1 -> Dot Product55/1(In1)
  delayMatch319/1 -> mul_Dot Product10_dotp_10/1(In1)
  mul_Dot Product11_dotp_9/1(Out1) -> delayMatch367/1
  delayMatch220/1 -> Dot Product612/1(In1)
  delayMatch322/1 -> mul_Dot Product10_dotp_7/1(In1)
  delayMatch326/1 -> mul_Dot Product10_dotp_3/1(In1)
  delayMatch47/1 -> mul_Dot Product1_dotp_12/1(In1)
  delayMatch283/1 -> Dot Product815/1(In1)
  mul_Dot Product14_dotp_15/1(Out1) -> delayMatch463/1
  CrossIC/1 -> LC vectorized/3(x)
  delayMatch329/1 -> mul_Dot Product10_dotp_0/1(In1)
  t3/13 -> Mux4_out1_12_term12/1
  delayMatch117/1 -> mul_Dot Product3_dotp_2/1(In1)
  delayMatch300/1 -> Dot Product92/1(In1)
  t25/14 -> mul_Dot Product9_dotp_13/2(In2)
  t11/1 -> mul_Dot Product2_dotp_0/2(In2)
  t25/8 -> mul_Dot Product9_dotp_7/2(In2)
  t25/7 -> mul_Dot Product9_dotp_6/2(In2)
  mul_Dot Product_dotp_4/1(Out1) -> delayMatch32/1
  delayMatch56/1 -> mul_Dot Product1_dotp_3/1(In1)
  mul_Dot Product_dotp_13/1(Out1) -> delayMatch41/1
  delayMatch235/1 -> mul_Dot Product7_dotp_4/1(In1)
  delayMatch287/1 -> mul_Dot Product9_dotp_12/1(In1)
  delayMatch288/1 -> mul_Dot Product9_dotp_11/1(In1)
  mul_Dot Product9_dotp_6/1(Out1) -> delayMatch304/1
  t/1 -> user_out/1
  delayMatch289/1 -> mul_Dot Product9_dotp_10/1(In1)
  delayMatch291/1 -> mul_Dot Product9_dotp_8/1(In1)
  mul_Dot Product14_dotp_3/1(Out1) -> delayMatch451/1
  delayMatch295/1 -> mul_Dot Product9_dotp_4/1(In1)
  delayMatch280/1 -> Dot Product812/1(In1)
  delayMatch277/1 -> Dot Product89/1(In1)
  mul_Dot Product5_dotp_14/1(Out1) -> delayMatch192/1
  delayMatch271/1 -> Dot Product83/1(In1)
  delayMatch264/1 -> mul_Dot Product8_dotp_5/1(In1)
  delayMatch270/1 -> Dot Product82/1(In1)
  mul_Dot Product_dotp_9/1(Out1) -> delayMatch37/1
  t9/5 -> mul_Dot Product1_dotp_4/2(In2)
  t23/12 -> mul_Dot Product8_dotp_11/2(In2)
  delayMatch253/1 -> Dot Product715/1(In1)
  delayMatch256/1 -> mul_Dot Product8_dotp_13/1(In1)
  t7/14 -> mul_Dot Product_dotp_13/2(In2)
  mul_Dot Product5_dotp_5/1(Out1) -> delayMatch183/1
  delayMatch257/1 -> mul_Dot Product8_dotp_12/1(In1)
  delayMatch261/1 -> mul_Dot Product8_dotp_8/1(In1)
  delayMatch177/1 -> mul_Dot Product5_dotp_2/1(In1)
  delayMatch262/1 -> mul_Dot Product8_dotp_7/1(In1)
  mul_Dot Product7_dotp_3/1(Out1) -> delayMatch241/1
  delayMatch265/1 -> mul_Dot Product8_dotp_4/1(In1)
  delayMatch266/1 -> mul_Dot Product8_dotp_3/1(In1)
  t3/15 -> Mux4_out1_14_term14/1
  delayMatch68/1 -> Dot Product114/1(In1)
  delayMatch267/1 -> mul_Dot Product8_dotp_2/1(In1)
  delayMatch250/1 -> Dot Product712/1(In1)
  delayMatch125/1 -> Dot Product37/1(In1)
  delayMatch59/1 -> mul_Dot Product1_dotp_0/1(In1)
  Selector14/1 -> t34/1
  delayMatch247/1 -> Dot Product79/1(In1)
  delayMatch245/1 -> Dot Product77/1(In1)
  t17/5 -> mul_Dot Product5_dotp_4/2(In2)
  t21/4 -> mul_Dot Product7_dotp_3/2(In2)
  delayMatch242/1 -> Dot Product74/1(In1)
  mul_Dot Product7_dotp_10/1(Out1) -> delayMatch248/1
  delayMatch241/1 -> Dot Product73/1(In1)
  mul_Dot Product14_dotp_7/1(Out1) -> delayMatch455/1
  t21/13 -> mul_Dot Product7_dotp_12/2(In2)
  t17/6 -> mul_Dot Product5_dotp_5/2(In2)
  t21/3 -> mul_Dot Product7_dotp_2/2(In2)
  delayMatch225/1 -> mul_Dot Product7_dotp_14/1(In1)
  delayMatch226/1 -> mul_Dot Product7_dotp_13/1(In1)
  delayMatch231/1 -> mul_Dot Product7_dotp_8/1(In1)
  delayMatch233/1 -> mul_Dot Product7_dotp_6/1(In1)
  delayMatch119/1 -> mul_Dot Product3_dotp_0/1(In1)
  delayMatch223/1 -> Dot Product615/1(In1)
  delayMatch212/1 -> Dot Product64/1(In1)
  delayMatch210/1 -> Dot Product62/1(In1)
  delayMatch3/1 -> mux2/6
  t19/12 -> mul_Dot Product6_dotp_11/2(In2)
  t15/7 -> mul_Dot Product4_dotp_6/2(In2)
  t19/10 -> mul_Dot Product6_dotp_9/2(In2)
  t19/9 -> mul_Dot Product6_dotp_8/2(In2)
  t19/8 -> mul_Dot Product6_dotp_7/2(In2)
  t19/1 -> mul_Dot Product6_dotp_0/2(In2)
  delayMatch194/1 -> mul_Dot Product6_dotp_15/1(In1)
  delayMatch196/1 -> mul_Dot Product6_dotp_13/1(In1)
  delayMatch197/1 -> mul_Dot Product6_dotp_12/1(In1)
  delayMatch202/1 -> mul_Dot Product6_dotp_7/1(In1)
  delayMatch94/1 -> Dot Product26/1(In1)
  mul_Dot Product12_dotp_6/1(Out1) -> delayMatch394/1
  delayMatch209/1 -> mul_Dot Product6_dotp_0/1(In1)
  delayMatch193/1 -> Dot Product515/1(In1)
  delayMatch192/1 -> Dot Product514/1(In1)
  delayMatch191/1 -> Dot Product513/1(In1)
  delayMatch185/1 -> Dot Product57/1(In1)
  delayMatch182/1 -> Dot Product54/1(In1)
  delayMatch181/1 -> Dot Product53/1(In1)
  delayMatch180/1 -> Dot Product52/1(In1)
  t17/4 -> mul_Dot Product5_dotp_3/2(In2)
  t17/1 -> mul_Dot Product5_dotp_0/2(In2)
  delayMatch370/1 -> Dot Product1121/1(In1)
  delayMatch172/1 -> mul_Dot Product5_dotp_7/1(In1)
  delayMatch175/1 -> mul_Dot Product5_dotp_4/1(In1)
  delayMatch176/1 -> mul_Dot Product5_dotp_3/1(In1)
  delayMatch31/1 -> Dot Product2/1(In1)
  delayMatch160/1 -> Dot Product412/1(In1)
  t9/1 -> mul_Dot Product1_dotp_0/2(In2)
  delayMatch158/1 -> Dot Product410/1(In1)
  delayMatch150/1 -> Dot Product42/1(In1)
  t15/10 -> mul_Dot Product4_dotp_9/2(In2)
  t15/6 -> mul_Dot Product4_dotp_5/2(In2)
  t15/5 -> mul_Dot Product4_dotp_4/2(In2)
  delayMatch116/1 -> mul_Dot Product3_dotp_3/1(In1)
  delayMatch138/1 -> mul_Dot Product4_dotp_11/1(In1)
  delayMatch146/1 -> mul_Dot Product4_dotp_3/1(In1)
  t7/4 -> mul_Dot Product_dotp_3/2(In2)
  delayMatch143/1 -> mul_Dot Product4_dotp_6/1(In1)
  mul_Dot Product6_dotp_13/1(Out1) -> delayMatch221/1
  delayMatch29/1 -> mul_Dot Product_dotp_0/1(In1)
  t7/2 -> mul_Dot Product_dotp_1/2(In2)
  delayMatch144/1 -> mul_Dot Product4_dotp_5/1(In1)
  t3/9 -> Mux4_out1_8_term8/1
  delayMatch132/1 -> Dot Product314/1(In1)
  mul_Dot Product3_dotp_12/1(Out1) -> delayMatch130/1
  delayMatch128/1 -> Dot Product310/1(In1)
  mul_Dot Product12_dotp_12/1(Out1) -> delayMatch400/1
  delayMatch123/1 -> Dot Product35/1(In1)
  t13/7 -> mul_Dot Product3_dotp_6/2(In2)
  t13/5 -> mul_Dot Product3_dotp_4/2(In2)
  t11/3 -> mul_Dot Product2_dotp_2/2(In2)
  t13/2 -> mul_Dot Product3_dotp_1/2(In2)
  delayMatch107/1 -> mul_Dot Product3_dotp_12/1(In1)
  delayMatch109/1 -> mul_Dot Product3_dotp_10/1(In1)
  delayMatch13/1 -> mux2/16
  delayMatch110/1 -> mul_Dot Product3_dotp_9/1(In1)
  delayMatch114/1 -> mul_Dot Product3_dotp_5/1(In1)
  delayMatch118/1 -> mul_Dot Product3_dotp_1/1(In1)
  delayMatch90/1 -> Dot Product22/1(In1)
  t11/14 -> mul_Dot Product2_dotp_13/2(In2)
  t11/5 -> mul_Dot Product2_dotp_4/2(In2)
  delayMatch76/1 -> mul_Dot Product2_dotp_13/1(In1)
  delayMatch77/1 -> mul_Dot Product2_dotp_12/1(In1)
  delayMatch78/1 -> mul_Dot Product2_dotp_11/1(In1)
  delayMatch83/1 -> mul_Dot Product2_dotp_6/1(In1)
  mul_Dot Product3_dotp_14/1(Out1) -> delayMatch132/1
  delayMatch85/1 -> mul_Dot Product2_dotp_4/1(In1)
  delayMatch86/1 -> mul_Dot Product2_dotp_3/1(In1)
  delayMatch87/1 -> mul_Dot Product2_dotp_2/1(In1)
  delayMatch67/1 -> Dot Product113/1(In1)
  delayMatch61/1 -> Dot Product17/1(In1)
  Demux_mux_1/1 -> LC vectorized/5(vi_in)
  delayMatch60/1 -> Dot Product16/1(In1)
  t9/15 -> mul_Dot Product1_dotp_14/2(In2)
  t9/10 -> mul_Dot Product1_dotp_9/2(In2)
  delayMatch15/1 -> mul_Dot Product_dotp_14/1(In1)
  t9/9 -> mul_Dot Product1_dotp_8/2(In2)
  delayMatch44/1 -> mul_Dot Product1_dotp_15/1(In1)
  delayMatch45/1 -> mul_Dot Product1_dotp_14/1(In1)
  delayMatch39/1 -> Dot Product10/1(In1)
  t3/1 -> Demux_mux_1/1
  delayMatch37/1 -> Dot Product8/1(In1)
  t7/8 -> mul_Dot Product_dotp_7/2(In2)
  t7/7 -> mul_Dot Product_dotp_6/2(In2)
  delayMatch20/1 -> mul_Dot Product_dotp_9/1(In1)
  Selector8/1 -> t22/1
  delayMatch23/1 -> mul_Dot Product_dotp_6/1(In1)
  mul_Dot Product13_dotp_5/1(Out1) -> delayMatch423/1
  delayMatch25/1 -> mul_Dot Product_dotp_4/1(In1)
  delayMatch28/1 -> mul_Dot Product_dotp_1/1(In1)
  delayMatch494/1 -> Index Vector/1
  delayMatch9/1 -> mux2/12
  delayMatch7/1 -> mux2/10
  delayMatch6/1 -> mux2/9
  t4/2 -> mux2/2
  t4/1 -> mux2/1
  t3/8 -> Mux4_out1_7_term7/1
  t3/6 -> Mux4_out1_5_term5/1
  t3/4 -> Demux_mux_1/4
  t3/2 -> Demux_mux_1/2
  Selector2/1 -> t10/1
  Compare To Constant/1(y) -> Delay_Switch/2
  in3_repeat1/1 -> crp_out_delay/1
  in1_repeat/1 -> t2/1
  PWM Generator/1(gup) -> Data Type Conversion1/1
  out_start_range/1 -> in4_repeat/1
  in/1 -> in2_repeat/1
  gate/1 -> in1_repeat/1
  Counter Free-Running/1(y) -> delayMatch496/1, in3_repeat/1
  mul_Dot Product1_dotp_15/1(Out1) -> delayMatch73/1
  mul_Dot Product1_dotp_13/1(Out1) -> delayMatch71/1
  mul_Dot Product1_dotp_6/1(Out1) -> delayMatch64/1
  mul_Dot Product11_dotp_15/1(Out1) -> delayMatch373/1
  mul_Dot Product1_dotp_10/1(Out1) -> delayMatch68/1
  mul_Dot Product12_dotp_15/1(Out1) -> delayMatch403/1
  mul_Dot Product13_dotp_4/1(Out1) -> delayMatch422/1
  mul_Dot Product1_dotp_8/1(Out1) -> delayMatch66/1
  mul_Dot Product4_dotp_4/1(Out1) -> delayMatch152/1
  delayMatch339/1 -> Dot Product1011/1(In1)
  mul_Dot Product1_dotp_5/1(Out1) -> delayMatch63/1
  mul_Dot Product1_dotp_14/1(Out1) -> delayMatch72/1
  mul_Dot Product10_dotp_11/1(Out1) -> delayMatch339/1
  mul_Dot Product_dotp_10/1(Out1) -> delayMatch38/1
  mul_Dot Product_dotp_11/1(Out1) -> delayMatch39/1
  mul_Dot Product10_dotp_5/1(Out1) -> delayMatch333/1
  mul_Dot Product4_dotp_11/1(Out1) -> delayMatch159/1
  mul_Dot Product6_dotp_3/1(Out1) -> delayMatch211/1
  delayMatch429/1 -> Dot Product1311/1(In1)
  mul_Dot Product_dotp_8/1(Out1) -> delayMatch36/1
  mul_Dot Product2_dotp_6/1(Out1) -> delayMatch94/1
  mul_Dot Product12_dotp_5/1(Out1) -> delayMatch393/1
  mul_Dot Product10_dotp_3/1(Out1) -> delayMatch331/1
  delayMatch189/1 -> Dot Product511/1(In1)
  mul_Dot Product10_dotp_8/1(Out1) -> delayMatch336/1
  mul_Dot Product10_dotp_9/1(Out1) -> delayMatch337/1
  mul_Dot Product11_dotp_10/1(Out1) -> delayMatch368/1
  mul_Dot Product7_dotp_5/1(Out1) -> delayMatch243/1
  mul_Dot Product6_dotp_5/1(Out1) -> delayMatch213/1
  mul_Dot Product9_dotp_10/1(Out1) -> delayMatch308/1
  mul_Dot Product11_dotp_7/1(Out1) -> delayMatch365/1
  mul_Dot Product11_dotp_12/1(Out1) -> delayMatch370/1
  mul_Dot Product12_dotp_13/1(Out1) -> delayMatch401/1
  mul_Dot Product12_dotp_7/1(Out1) -> delayMatch395/1
  mul_Dot Product3_dotp_6/1(Out1) -> delayMatch124/1
  mul_Dot Product12_dotp_8/1(Out1) -> delayMatch396/1
  mul_Dot Product12_dotp_9/1(Out1) -> delayMatch397/1
  mul_Dot Product3_dotp_4/1(Out1) -> delayMatch122/1
  mul_Dot Product13_dotp_10/1(Out1) -> delayMatch428/1
  mul_Dot Product5_dotp_11/1(Out1) -> delayMatch189/1
  mul_Dot Product13_dotp_11/1(Out1) -> delayMatch429/1
  mul_Dot Product8_dotp_13/1(Out1) -> delayMatch281/1
  mul_Dot Product13_dotp_12/1(Out1) -> delayMatch430/1
  delayMatch452/1 -> Dot Product144/1(In1)
  mul_Dot Product9_dotp_11/1(Out1) -> delayMatch309/1
  mul_Dot Product13_dotp_8/1(Out1) -> delayMatch426/1
  mul_Dot Product14_dotp_11/1(Out1) -> delayMatch459/1
  mul_Dot Product9_dotp_9/1(Out1) -> delayMatch307/1
  mul_Dot Product14_dotp_13/1(Out1) -> delayMatch461/1
  mul_Dot Product14_dotp_14/1(Out1) -> delayMatch462/1
  mul_Dot Product7_dotp_8/1(Out1) -> delayMatch246/1
  mul_Dot Product14_dotp_5/1(Out1) -> delayMatch453/1
  mul_Dot Product14_dotp_6/1(Out1) -> delayMatch454/1
  mul_Dot Product14_dotp_8/1(Out1) -> delayMatch456/1
  mul_Dot Product9_dotp_8/1(Out1) -> delayMatch306/1
  mul_Dot Product15_dotp_10/1(Out1) -> delayMatch488/1
  mul_Dot Product4_dotp_15/1(Out1) -> delayMatch163/1
  mul_Dot Product2_dotp_13/1(Out1) -> delayMatch101/1
  mul_Dot Product15_dotp_14/1(Out1) -> delayMatch492/1
  mul_Dot Product4_dotp_9/1(Out1) -> delayMatch157/1
  delayMatch337/1 -> Dot Product109/1(In1)
  mul_Dot Product15_dotp_3/1(Out1) -> delayMatch481/1
  mul_Dot Product15_dotp_4/1(Out1) -> delayMatch482/1
  mul_Dot Product15_dotp_5/1(Out1) -> delayMatch483/1
  delayMatch310/1 -> Dot Product912/1(In1)
  mul_Dot Product15_dotp_7/1(Out1) -> delayMatch485/1
  mul_Dot Product8_dotp_4/1(Out1) -> delayMatch272/1
  mul_Dot Product8_dotp_10/1(Out1) -> delayMatch278/1
  mul_Dot Product15_dotp_8/1(Out1) -> delayMatch486/1
  mul_Dot Product2_dotp_10/1(Out1) -> delayMatch98/1
  mul_Dot Product2_dotp_12/1(Out1) -> delayMatch100/1
  mul_Dot Product2_dotp_9/1(Out1) -> delayMatch97/1
  mul_Dot Product5_dotp_15/1(Out1) -> delayMatch193/1
  mul_Dot Product2_dotp_14/1(Out1) -> delayMatch102/1
  delayMatch301/1 -> Dot Product93/1(In1)
  mul_Dot Product3_dotp_15/1(Out1) -> delayMatch133/1
  mul_Dot Product2_dotp_4/1(Out1) -> delayMatch92/1
  mul_Dot Product3_dotp_10/1(Out1) -> delayMatch128/1
  mul_Dot Product3_dotp_11/1(Out1) -> delayMatch129/1
  delayMatch308/1 -> Dot Product910/1(In1)
  mul_Dot Product3_dotp_5/1(Out1) -> delayMatch123/1
  mul_Dot Product3_dotp_7/1(Out1) -> delayMatch125/1
  delayMatch458/1 -> Dot Product1410/1(In1)
  mul_Dot Product4_dotp_10/1(Out1) -> delayMatch158/1
  delayMatch187/1 -> Dot Product59/1(In1)
  mul_Dot Product4_dotp_12/1(Out1) -> delayMatch160/1
  mul_Dot Product4_dotp_8/1(Out1) -> delayMatch156/1
  mul_Dot Product6_dotp_11/1(Out1) -> delayMatch219/1
  From/1 -> t4/1
  mul_Dot Product6_dotp_15/1(Out1) -> delayMatch223/1
  mul_Dot Product6_dotp_8/1(Out1) -> delayMatch216/1
  mul_Dot Product7_dotp_12/1(Out1) -> delayMatch250/1
  mul_Dot Product7_dotp_13/1(Out1) -> delayMatch251/1
  delayMatch365/1 -> Dot Product1116/1(In1)
  mul_Dot Product7_dotp_7/1(Out1) -> delayMatch245/1
  mul_Dot Product8_dotp_11/1(Out1) -> delayMatch279/1
  mul_Dot Product8_dotp_15/1(Out1) -> delayMatch283/1
  mul_Dot Product8_dotp_3/1(Out1) -> delayMatch271/1
  mul_Dot Product8_dotp_6/1(Out1) -> delayMatch274/1
  mul_Dot Product8_dotp_7/1(Out1) -> delayMatch275/1
  mul_Dot Product9_dotp_13/1(Out1) -> delayMatch311/1
  delayMatch186/1 -> Dot Product58/1(In1)
  mul_Dot Product9_dotp_7/1(Out1) -> delayMatch305/1
  delayMatch394/1 -> Dot Product126/1(In1)
  delayMatch423/1 -> Dot Product135/1(In1)
  delayMatch273/1 -> Dot Product85/1(In1)
  delayMatch484/1 -> Dot Product156/1(In1)
  delayMatch335/1 -> Dot Product107/1(In1)
  delayMatch336/1 -> Dot Product108/1(In1)
  delayMatch276/1 -> Dot Product88/1(In1)
  delayMatch426/1 -> Dot Product138/1(In1)
  delayMatch459/1 -> Dot Product1411/1(In1)
  delayMatch95/1 -> Dot Product27/1(In1)
  delayMatch460/1 -> Dot Product1412/1(In1)
  delayMatch400/1 -> Dot Product1212/1(In1)
  delayMatch341/1 -> Dot Product1013/1(In1)
  Selector/1 -> t6/1
